simulink model "gm_mandelbrot_fpga"  (R2019b)
settings: Solver=FixedStepDiscrete  StartTime=0.0  StopTime=33.5e-3  FixedStep=0.5*Ts  RelTol=1e-3  EnableMultiTasking=on
undefined symbols (not defined in the file or in its folder): BUTTON_CLOCK_DIV, BUTTON_DEBOUNCE, BUTTON_POLLING, LUT_BLUE, LUT_GREEN, LUT_RED, MAX_ITERATIONS, PIXEL_TIME, TRASLATION_FACTOR, Ts, VGA_HORIZONTAL_BACK_PORCH, VGA_HORIZONTAL_FRONT_PORCH, VGA_HORIZONTAL_RESOLUTION, VGA_HORIZONTAL_SYNC, VGA_VERTICAL_BACK_PORCH, VGA_VERTICAL_FRONT_PORCH, VGA_VERTICAL_RESOLUTION, VGA_VERTICAL_SYNC, ZOOM_FACTOR
libraries: simulink x132, hdlsllib x20, visionsinks x1
(part 2 of 9)

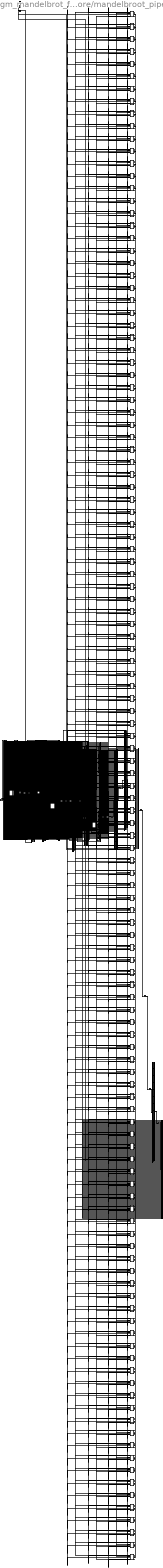
== system gm_mandelbrot_fpga/mandelbrot_top/mandelbrot_core/mandelbroot_pipeline ==
  c : Inport  OutDataTypeStr=fixdt(1, 18, 15)  PortDimensions=1  SampleTime=1.35e-08
      settings: SignalType=complex
  Constant : Constant  Value=0  OutDataTypeStr=boolean  SampleTime=-1
  Constant2 : Constant  Value=127  OutDataTypeStr=fixdt(0, 7, 0)  SampleTime=-1
  Delay{,1..3} (4 alike) : Delay  DelayLength=double(1)  InitialCondition=0  SampleTime=1.35e-08
  Demux1_mux_1 : Mux  Inputs=127
  Demux2_mux_1 : Mux  Inputs=127
  Demux3_mux_1 : Mux  Inputs=127
  Demux_mux_1 : Mux  Inputs=127
  Signal Specification : SignalSpecification  OutDataTypeStr=boolean  Dimensions=128
  Signal Specification1 : SignalSpecification  OutDataTypeStr=fixdt(1, 18, 15)  Dimensions=128
  Signal Specification2 : SignalSpecification  OutDataTypeStr=fixdt(1, 18, 15)  Dimensions=128
  Signal Specification3 : SignalSpecification  OutDataTypeStr=fixdt(0, 7, 0)  Dimensions=128
  Signal Specification4 : SignalSpecification  OutDataTypeStr=boolean  Dimensions=127
  Signal Specification5 : SignalSpecification  OutDataTypeStr=fixdt(1, 18, 15)  Dimensions=127
  Signal Specification6 : SignalSpecification  OutDataTypeStr=fixdt(1, 18, 15)  Dimensions=127
  Signal Specification7 : SignalSpecification  OutDataTypeStr=fixdt(0, 7, 0)  Dimensions=127
  Terminator : Terminator
  Terminator1 : Terminator
  Terminator2 : Terminator
  concatenate{,1..3} (4 alike) : Concatenate  NumInputs=128
  mandelbroot_array_instance1 : Subsystem
  mandelbroot_array_instance10 : Subsystem
  mandelbroot_array_instance100 : Subsystem
  mandelbroot_array_instance101 : Subsystem
  mandelbroot_array_instance102 : Subsystem
  mandelbroot_array_instance103 : Subsystem
  mandelbroot_array_instance104 : Subsystem
  mandelbroot_array_instance105 : Subsystem
  mandelbroot_array_instance106 : Subsystem
  mandelbroot_array_instance107 : Subsystem
  mandelbroot_array_instance108 : Subsystem
  mandelbroot_array_instance109 : Subsystem
  mandelbroot_array_instance11 : Subsystem
  mandelbroot_array_instance110 : Subsystem
  mandelbroot_array_instance111 : Subsystem
  mandelbroot_array_instance112 : Subsystem
  mandelbroot_array_instance113 : Subsystem
  mandelbroot_array_instance114 : Subsystem
  mandelbroot_array_instance115 : Subsystem
  mandelbroot_array_instance116 : Subsystem
  mandelbroot_array_instance117 : Subsystem
  mandelbroot_array_instance118 : Subsystem
  mandelbroot_array_instance119 : Subsystem
  mandelbroot_array_instance12 : Subsystem
  mandelbroot_array_instance120 : Subsystem
  mandelbroot_array_instance121 : Subsystem
  mandelbroot_array_instance122 : Subsystem
  mandelbroot_array_instance123 : Subsystem
  mandelbroot_array_instance124 : Subsystem
  mandelbroot_array_instance125 : Subsystem
  mandelbroot_array_instance126 : Subsystem
  mandelbroot_array_instance127 : Subsystem
  mandelbroot_array_instance128 : Subsystem
  mandelbroot_array_instance13 : Subsystem
  mandelbroot_array_instance14 : Subsystem
  mandelbroot_array_instance15 : Subsystem
  mandelbroot_array_instance16 : Subsystem
  mandelbroot_array_instance17 : Subsystem
  mandelbroot_array_instance18 : Subsystem
  mandelbroot_array_instance19 : Subsystem
  mandelbroot_array_instance2 : Subsystem
  mandelbroot_array_instance20 : Subsystem
  mandelbroot_array_instance21 : Subsystem
  mandelbroot_array_instance22 : Subsystem
  mandelbroot_array_instance23 : Subsystem
  mandelbroot_array_instance24 : Subsystem
  mandelbroot_array_instance25 : Subsystem
  mandelbroot_array_instance26 : Subsystem
  mandelbroot_array_instance27 : Subsystem
  mandelbroot_array_instance28 : Subsystem
  mandelbroot_array_instance29 : Subsystem
  mandelbroot_array_instance3 : Subsystem
  mandelbroot_array_instance30 : Subsystem
  mandelbroot_array_instance31 : Subsystem
  mandelbroot_array_instance32 : Subsystem
  mandelbroot_array_instance33 : Subsystem
  mandelbroot_array_instance34 : Subsystem
  mandelbroot_array_instance35 : Subsystem
  mandelbroot_array_instance36 : Subsystem
  mandelbroot_array_instance37 : Subsystem
  mandelbroot_array_instance38 : Subsystem
  mandelbroot_array_instance39 : Subsystem
  mandelbroot_array_instance4 : Subsystem
  mandelbroot_array_instance40 : Subsystem
  mandelbroot_array_instance41 : Subsystem
  mandelbroot_array_instance42 : Subsystem
  mandelbroot_array_instance43 : Subsystem
  mandelbroot_array_instance44 : Subsystem
  mandelbroot_array_instance45 : Subsystem
  mandelbroot_array_instance46 : Subsystem
  mandelbroot_array_instance47 : Subsystem
  mandelbroot_array_instance48 : Subsystem
  mandelbroot_array_instance49 : Subsystem
  mandelbroot_array_instance5 : Subsystem
  mandelbroot_array_instance50 : Subsystem
  mandelbroot_array_instance51 : Subsystem
  mandelbroot_array_instance52 : Subsystem
  mandelbroot_array_instance53 : Subsystem
  mandelbroot_array_instance54 : Subsystem
  mandelbroot_array_instance55 : Subsystem
  mandelbroot_array_instance56 : Subsystem
  mandelbroot_array_instance57 : Subsystem
  mandelbroot_array_instance58 : Subsystem
  mandelbroot_array_instance59 : Subsystem
  mandelbroot_array_instance6 : Subsystem
  mandelbroot_array_instance60 : Subsystem
  mandelbroot_array_instance61 : Subsystem
  mandelbroot_array_instance62 : Subsystem
  mandelbroot_array_instance63 : Subsystem
  mandelbroot_array_instance64 : Subsystem
  mandelbroot_array_instance65 : Subsystem
  mandelbroot_array_instance66 : Subsystem
  mandelbroot_array_instance67 : Subsystem
  mandelbroot_array_instance68 : Subsystem
  mandelbroot_array_instance69 : Subsystem
  mandelbroot_array_instance7 : Subsystem
  mandelbroot_array_instance70 : Subsystem
  mandelbroot_array_instance71 : Subsystem
  mandelbroot_array_instance72 : Subsystem
  mandelbroot_array_instance73 : Subsystem
  mandelbroot_array_instance74 : Subsystem
  mandelbroot_array_instance75 : Subsystem
  mandelbroot_array_instance76 : Subsystem
  mandelbroot_array_instance77 : Subsystem
  mandelbroot_array_instance78 : Subsystem
  mandelbroot_array_instance79 : Subsystem
  mandelbroot_array_instance8 : Subsystem
  mandelbroot_array_instance80 : Subsystem
  mandelbroot_array_instance81 : Subsystem
  mandelbroot_array_instance82 : Subsystem
  mandelbroot_array_instance83 : Subsystem
  mandelbroot_array_instance84 : Subsystem
  mandelbroot_array_instance85 : Subsystem
  mandelbroot_array_instance86 : Subsystem
  mandelbroot_array_instance87 : Subsystem
  mandelbroot_array_instance88 : Subsystem
  mandelbroot_array_instance89 : Subsystem
  mandelbroot_array_instance9 : Subsystem
  mandelbroot_array_instance90 : Subsystem
  mandelbroot_array_instance91 : Subsystem
  mandelbroot_array_instance92 : Subsystem
  mandelbroot_array_instance93 : Subsystem
  mandelbroot_array_instance94 : Subsystem
  mandelbroot_array_instance95 : Subsystem
  mandelbroot_array_instance96 : Subsystem
  mandelbroot_array_instance97 : Subsystem
  mandelbroot_array_instance98 : Subsystem
  mandelbroot_array_instance99 : Subsystem
  t{,1..3,12..15} (8 alike) : Demux  Outputs=128
  t{4,6,8,10} (4 alike) : Concatenate  NumInputs=128
  t{5,7,9,11} (4 alike) : Reshape
  t{16..19} (4 alike) : Demux  Outputs=127
  result : Outport  VectorParamsAs1DForOutWhenUnconnected=off
  wires:
  c/1 -> concatenate2/1, concatenate/1
  Constant/1 -> concatenate1/1
  Constant2/1 -> concatenate3/1
  Delay/1 -> Signal Specification/1
  Delay1/1 -> Signal Specification1/1
  Delay2/1 -> Signal Specification3/1
  Delay3/1 -> Signal Specification2/1
  Demux_mux_1/1 -> Signal Specification4/1
  Demux1_mux_1/1 -> Signal Specification5/1
  Demux2_mux_1/1 -> Signal Specification6/1
  Demux3_mux_1/1 -> Signal Specification7/1
  Signal Specification/1 -> t12/1
  Signal Specification1/1 -> t13/1
  Signal Specification2/1 -> t14/1
  Signal Specification3/1 -> t15/1
  Signal Specification4/1 -> t17/1
  Signal Specification5/1 -> t18/1
  Signal Specification6/1 -> t16/1
  Signal Specification7/1 -> t19/1
  concatenate/1 -> t2/1
  concatenate1/1 -> t/1
  concatenate2/1 -> t1/1
  concatenate3/1 -> t3/1
  t5/1 -> Delay/1
  t7/1 -> Delay1/1
  t9/1 -> Delay3/1
  t11/1 -> Delay2/1
  t/1 -> mandelbroot_array_instance1/1(stop_in)
  t/2 -> mandelbroot_array_instance2/1(stop_in)
  t/3 -> mandelbroot_array_instance3/1(stop_in)
  t/4 -> mandelbroot_array_instance4/1(stop_in)
  t/5 -> mandelbroot_array_instance5/1(stop_in)
  t/6 -> mandelbroot_array_instance6/1(stop_in)
  t/7 -> mandelbroot_array_instance7/1(stop_in)
  t/8 -> mandelbroot_array_instance8/1(stop_in)
  t/9 -> mandelbroot_array_instance9/1(stop_in)
  t/10 -> mandelbroot_array_instance10/1(stop_in)
  t/11 -> mandelbroot_array_instance11/1(stop_in)
  t/12 -> mandelbroot_array_instance12/1(stop_in)
  t/13 -> mandelbroot_array_instance13/1(stop_in)
  t/14 -> mandelbroot_array_instance14/1(stop_in)
  t/15 -> mandelbroot_array_instance15/1(stop_in)
  t/16 -> mandelbroot_array_instance16/1(stop_in)
  t/17 -> mandelbroot_array_instance17/1(stop_in)
  t/18 -> mandelbroot_array_instance18/1(stop_in)
  t/19 -> mandelbroot_array_instance19/1(stop_in)
  t/20 -> mandelbroot_array_instance20/1(stop_in)
  t/21 -> mandelbroot_array_instance21/1(stop_in)
  t/22 -> mandelbroot_array_instance22/1(stop_in)
  t/23 -> mandelbroot_array_instance23/1(stop_in)
  t/24 -> mandelbroot_array_instance24/1(stop_in)
  t/25 -> mandelbroot_array_instance25/1(stop_in)
  t/26 -> mandelbroot_array_instance26/1(stop_in)
  t/27 -> mandelbroot_array_instance27/1(stop_in)
  t/28 -> mandelbroot_array_instance28/1(stop_in)
  t/29 -> mandelbroot_array_instance29/1(stop_in)
  t/30 -> mandelbroot_array_instance30/1(stop_in)
  t/31 -> mandelbroot_array_instance31/1(stop_in)
  t/32 -> mandelbroot_array_instance32/1(stop_in)
  t/33 -> mandelbroot_array_instance33/1(stop_in)
  t/34 -> mandelbroot_array_instance34/1(stop_in)
  t/35 -> mandelbroot_array_instance35/1(stop_in)
  t/36 -> mandelbroot_array_instance36/1(stop_in)
  t/37 -> mandelbroot_array_instance37/1(stop_in)
  t/38 -> mandelbroot_array_instance38/1(stop_in)
  t/39 -> mandelbroot_array_instance39/1(stop_in)
  t/40 -> mandelbroot_array_instance40/1(stop_in)
  t/41 -> mandelbroot_array_instance41/1(stop_in)
  t/42 -> mandelbroot_array_instance42/1(stop_in)
  t/43 -> mandelbroot_array_instance43/1(stop_in)
  t/44 -> mandelbroot_array_instance44/1(stop_in)
  t/45 -> mandelbroot_array_instance45/1(stop_in)
  t/46 -> mandelbroot_array_instance46/1(stop_in)
  t/47 -> mandelbroot_array_instance47/1(stop_in)
  t/48 -> mandelbroot_array_instance48/1(stop_in)
  t/49 -> mandelbroot_array_instance49/1(stop_in)
  t/50 -> mandelbroot_array_instance50/1(stop_in)
  t/51 -> mandelbroot_array_instance51/1(stop_in)
  t/52 -> mandelbroot_array_instance52/1(stop_in)
  t/53 -> mandelbroot_array_instance53/1(stop_in)
  t/54 -> mandelbroot_array_instance54/1(stop_in)
  t/55 -> mandelbroot_array_instance55/1(stop_in)
  t/56 -> mandelbroot_array_instance56/1(stop_in)
  t/57 -> mandelbroot_array_instance57/1(stop_in)
  t/58 -> mandelbroot_array_instance58/1(stop_in)
  t/59 -> mandelbroot_array_instance59/1(stop_in)
  t/60 -> mandelbroot_array_instance60/1(stop_in)
  t/61 -> mandelbroot_array_instance61/1(stop_in)
  t/62 -> mandelbroot_array_instance62/1(stop_in)
  t/63 -> mandelbroot_array_instance63/1(stop_in)
  t/64 -> mandelbroot_array_instance64/1(stop_in)
  t/65 -> mandelbroot_array_instance65/1(stop_in)
  t/66 -> mandelbroot_array_instance66/1(stop_in)
  t/67 -> mandelbroot_array_instance67/1(stop_in)
  t/68 -> mandelbroot_array_instance68/1(stop_in)
  t/69 -> mandelbroot_array_instance69/1(stop_in)
  t/70 -> mandelbroot_array_instance70/1(stop_in)
  t/71 -> mandelbroot_array_instance71/1(stop_in)
  t/72 -> mandelbroot_array_instance72/1(stop_in)
  t/73 -> mandelbroot_array_instance73/1(stop_in)
  t/74 -> mandelbroot_array_instance74/1(stop_in)
  t/75 -> mandelbroot_array_instance75/1(stop_in)
  t/76 -> mandelbroot_array_instance76/1(stop_in)
  t/77 -> mandelbroot_array_instance77/1(stop_in)
  t/78 -> mandelbroot_array_instance78/1(stop_in)
  t/79 -> mandelbroot_array_instance79/1(stop_in)
  t/80 -> mandelbroot_array_instance80/1(stop_in)
  t/81 -> mandelbroot_array_instance81/1(stop_in)
  t/82 -> mandelbroot_array_instance82/1(stop_in)
  t/83 -> mandelbroot_array_instance83/1(stop_in)
  t/84 -> mandelbroot_array_instance84/1(stop_in)
  t/85 -> mandelbroot_array_instance85/1(stop_in)
  t/86 -> mandelbroot_array_instance86/1(stop_in)
  t/87 -> mandelbroot_array_instance87/1(stop_in)
  t/88 -> mandelbroot_array_instance88/1(stop_in)
  t/89 -> mandelbroot_array_instance89/1(stop_in)
  t/90 -> mandelbroot_array_instance90/1(stop_in)
  t/91 -> mandelbroot_array_instance91/1(stop_in)
  t/92 -> mandelbroot_array_instance92/1(stop_in)
  t/93 -> mandelbroot_array_instance93/1(stop_in)
  t/94 -> mandelbroot_array_instance94/1(stop_in)
  t/95 -> mandelbroot_array_instance95/1(stop_in)
  t/96 -> mandelbroot_array_instance96/1(stop_in)
  t/97 -> mandelbroot_array_instance97/1(stop_in)
  t/98 -> mandelbroot_array_instance98/1(stop_in)
  t/99 -> mandelbroot_array_instance99/1(stop_in)
  t/100 -> mandelbroot_array_instance100/1(stop_in)
  t/101 -> mandelbroot_array_instance101/1(stop_in)
  t/102 -> mandelbroot_array_instance102/1(stop_in)
  t/103 -> mandelbroot_array_instance103/1(stop_in)
  t/104 -> mandelbroot_array_instance104/1(stop_in)
  t/105 -> mandelbroot_array_instance105/1(stop_in)
  t/106 -> mandelbroot_array_instance106/1(stop_in)
  t/107 -> mandelbroot_array_instance107/1(stop_in)
  t/108 -> mandelbroot_array_instance108/1(stop_in)
  t/109 -> mandelbroot_array_instance109/1(stop_in)
  t/110 -> mandelbroot_array_instance110/1(stop_in)
  t/111 -> mandelbroot_array_instance111/1(stop_in)
  t/112 -> mandelbroot_array_instance112/1(stop_in)
  t/113 -> mandelbroot_array_instance113/1(stop_in)
  t/114 -> mandelbroot_array_instance114/1(stop_in)
  t/115 -> mandelbroot_array_instance115/1(stop_in)
  t/116 -> mandelbroot_array_instance116/1(stop_in)
  t/117 -> mandelbroot_array_instance117/1(stop_in)
  t/118 -> mandelbroot_array_instance118/1(stop_in)
  t/119 -> mandelbroot_array_instance119/1(stop_in)
  t/120 -> mandelbroot_array_instance120/1(stop_in)
  t/121 -> mandelbroot_array_instance121/1(stop_in)
  t/122 -> mandelbroot_array_instance122/1(stop_in)
  t/123 -> mandelbroot_array_instance123/1(stop_in)
  t/124 -> mandelbroot_array_instance124/1(stop_in)
  t/125 -> mandelbroot_array_instance125/1(stop_in)
  t/126 -> mandelbroot_array_instance126/1(stop_in)
  t/127 -> mandelbroot_array_instance127/1(stop_in)
  t/128 -> mandelbroot_array_instance128/1(stop_in)
  t1/1 -> mandelbroot_array_instance1/2(z_in)
  t1/2 -> mandelbroot_array_instance2/2(z_in)
  t1/3 -> mandelbroot_array_instance3/2(z_in)
  t1/4 -> mandelbroot_array_instance4/2(z_in)
  t1/5 -> mandelbroot_array_instance5/2(z_in)
  t1/6 -> mandelbroot_array_instance6/2(z_in)
  t1/7 -> mandelbroot_array_instance7/2(z_in)
  t1/8 -> mandelbroot_array_instance8/2(z_in)
  t1/9 -> mandelbroot_array_instance9/2(z_in)
  t1/10 -> mandelbroot_array_instance10/2(z_in)
  t1/11 -> mandelbroot_array_instance11/2(z_in)
  t1/12 -> mandelbroot_array_instance12/2(z_in)
  t1/13 -> mandelbroot_array_instance13/2(z_in)
  t1/14 -> mandelbroot_array_instance14/2(z_in)
  t1/15 -> mandelbroot_array_instance15/2(z_in)
  t1/16 -> mandelbroot_array_instance16/2(z_in)
  t1/17 -> mandelbroot_array_instance17/2(z_in)
  t1/18 -> mandelbroot_array_instance18/2(z_in)
  t1/19 -> mandelbroot_array_instance19/2(z_in)
  t1/20 -> mandelbroot_array_instance20/2(z_in)
  t1/21 -> mandelbroot_array_instance21/2(z_in)
  t1/22 -> mandelbroot_array_instance22/2(z_in)
  t1/23 -> mandelbroot_array_instance23/2(z_in)
  t1/24 -> mandelbroot_array_instance24/2(z_in)
  t1/25 -> mandelbroot_array_instance25/2(z_in)
  t1/26 -> mandelbroot_array_instance26/2(z_in)
  t1/27 -> mandelbroot_array_instance27/2(z_in)
  t1/28 -> mandelbroot_array_instance28/2(z_in)
  t1/29 -> mandelbroot_array_instance29/2(z_in)
  t1/30 -> mandelbroot_array_instance30/2(z_in)
  t1/31 -> mandelbroot_array_instance31/2(z_in)
  t1/32 -> mandelbroot_array_instance32/2(z_in)
  t1/33 -> mandelbroot_array_instance33/2(z_in)
  t1/34 -> mandelbroot_array_instance34/2(z_in)
  t1/35 -> mandelbroot_array_instance35/2(z_in)
  t1/36 -> mandelbroot_array_instance36/2(z_in)
  t1/37 -> mandelbroot_array_instance37/2(z_in)
  t1/38 -> mandelbroot_array_instance38/2(z_in)
  t1/39 -> mandelbroot_array_instance39/2(z_in)
  t1/40 -> mandelbroot_array_instance40/2(z_in)
  t1/41 -> mandelbroot_array_instance41/2(z_in)
  t1/42 -> mandelbroot_array_instance42/2(z_in)
  t1/43 -> mandelbroot_array_instance43/2(z_in)
  t1/44 -> mandelbroot_array_instance44/2(z_in)
  t1/45 -> mandelbroot_array_instance45/2(z_in)
  t1/46 -> mandelbroot_array_instance46/2(z_in)
  t1/47 -> mandelbroot_array_instance47/2(z_in)
  t1/48 -> mandelbroot_array_instance48/2(z_in)
  t1/49 -> mandelbroot_array_instance49/2(z_in)
  t1/50 -> mandelbroot_array_instance50/2(z_in)
  t1/51 -> mandelbroot_array_instance51/2(z_in)
  t1/52 -> mandelbroot_array_instance52/2(z_in)
  t1/53 -> mandelbroot_array_instance53/2(z_in)
  t1/54 -> mandelbroot_array_instance54/2(z_in)
  t1/55 -> mandelbroot_array_instance55/2(z_in)
  t1/56 -> mandelbroot_array_instance56/2(z_in)
  t1/57 -> mandelbroot_array_instance57/2(z_in)
  t1/58 -> mandelbroot_array_instance58/2(z_in)
  t1/59 -> mandelbroot_array_instance59/2(z_in)
  t1/60 -> mandelbroot_array_instance60/2(z_in)
  t1/61 -> mandelbroot_array_instance61/2(z_in)
  t1/62 -> mandelbroot_array_instance62/2(z_in)
  t1/63 -> mandelbroot_array_instance63/2(z_in)
  t1/64 -> mandelbroot_array_instance64/2(z_in)
  t1/65 -> mandelbroot_array_instance65/2(z_in)
  t1/66 -> mandelbroot_array_instance66/2(z_in)
  t1/67 -> mandelbroot_array_instance67/2(z_in)
  t1/68 -> mandelbroot_array_instance68/2(z_in)
  t1/69 -> mandelbroot_array_instance69/2(z_in)
  t1/70 -> mandelbroot_array_instance70/2(z_in)
  t1/71 -> mandelbroot_array_instance71/2(z_in)
  t1/72 -> mandelbroot_array_instance72/2(z_in)
  t1/73 -> mandelbroot_array_instance73/2(z_in)
  t1/74 -> mandelbroot_array_instance74/2(z_in)
  t1/75 -> mandelbroot_array_instance75/2(z_in)
  t1/76 -> mandelbroot_array_instance76/2(z_in)
  t1/77 -> mandelbroot_array_instance77/2(z_in)
  t1/78 -> mandelbroot_array_instance78/2(z_in)
  t1/79 -> mandelbroot_array_instance79/2(z_in)
  t1/80 -> mandelbroot_array_instance80/2(z_in)
  t1/81 -> mandelbroot_array_instance81/2(z_in)
  t1/82 -> mandelbroot_array_instance82/2(z_in)
  t1/83 -> mandelbroot_array_instance83/2(z_in)
  t1/84 -> mandelbroot_array_instance84/2(z_in)
  t1/85 -> mandelbroot_array_instance85/2(z_in)
  t1/86 -> mandelbroot_array_instance86/2(z_in)
  t1/87 -> mandelbroot_array_instance87/2(z_in)
  t1/88 -> mandelbroot_array_instance88/2(z_in)
  t1/89 -> mandelbroot_array_instance89/2(z_in)
  t1/90 -> mandelbroot_array_instance90/2(z_in)
  t1/91 -> mandelbroot_array_instance91/2(z_in)
  t1/92 -> mandelbroot_array_instance92/2(z_in)
  t1/93 -> mandelbroot_array_instance93/2(z_in)
  t1/94 -> mandelbroot_array_instance94/2(z_in)
  t1/95 -> mandelbroot_array_instance95/2(z_in)
  t1/96 -> mandelbroot_array_instance96/2(z_in)
  t1/97 -> mandelbroot_array_instance97/2(z_in)
  t1/98 -> mandelbroot_array_instance98/2(z_in)
  t1/99 -> mandelbroot_array_instance99/2(z_in)
  t1/100 -> mandelbroot_array_instance100/2(z_in)
  t1/101 -> mandelbroot_array_instance101/2(z_in)
  t1/102 -> mandelbroot_array_instance102/2(z_in)
  t1/103 -> mandelbroot_array_instance103/2(z_in)
  t1/104 -> mandelbroot_array_instance104/2(z_in)
  t1/105 -> mandelbroot_array_instance105/2(z_in)
  t1/106 -> mandelbroot_array_instance106/2(z_in)
  t1/107 -> mandelbroot_array_instance107/2(z_in)
  t1/108 -> mandelbroot_array_instance108/2(z_in)
  t1/109 -> mandelbroot_array_instance109/2(z_in)
  t1/110 -> mandelbroot_array_instance110/2(z_in)
  t1/111 -> mandelbroot_array_instance111/2(z_in)
  t1/112 -> mandelbroot_array_instance112/2(z_in)
  t1/113 -> mandelbroot_array_instance113/2(z_in)
  t1/114 -> mandelbroot_array_instance114/2(z_in)
  t1/115 -> mandelbroot_array_instance115/2(z_in)
  t1/116 -> mandelbroot_array_instance116/2(z_in)
  t1/117 -> mandelbroot_array_instance117/2(z_in)
  t1/118 -> mandelbroot_array_instance118/2(z_in)
  t1/119 -> mandelbroot_array_instance119/2(z_in)
  t1/120 -> mandelbroot_array_instance120/2(z_in)
  t1/121 -> mandelbroot_array_instance121/2(z_in)
  t1/122 -> mandelbroot_array_instance122/2(z_in)
  t1/123 -> mandelbroot_array_instance123/2(z_in)
  t1/124 -> mandelbroot_array_instance124/2(z_in)
  t1/125 -> mandelbroot_array_instance125/2(z_in)
  t1/126 -> mandelbroot_array_instance126/2(z_in)
  t1/127 -> mandelbroot_array_instance127/2(z_in)
  t1/128 -> mandelbroot_array_instance128/2(z_in)
  t2/1 -> mandelbroot_array_instance1/3(c_in)
  t2/2 -> mandelbroot_array_instance2/3(c_in)
  t2/3 -> mandelbroot_array_instance3/3(c_in)
  t2/4 -> mandelbroot_array_instance4/3(c_in)
  t2/5 -> mandelbroot_array_instance5/3(c_in)
  t2/6 -> mandelbroot_array_instance6/3(c_in)
  t2/7 -> mandelbroot_array_instance7/3(c_in)
  t2/8 -> mandelbroot_array_instance8/3(c_in)
  t2/9 -> mandelbroot_array_instance9/3(c_in)
  t2/10 -> mandelbroot_array_instance10/3(c_in)
  t2/11 -> mandelbroot_array_instance11/3(c_in)
  t2/12 -> mandelbroot_array_instance12/3(c_in)
  t2/13 -> mandelbroot_array_instance13/3(c_in)
  t2/14 -> mandelbroot_array_instance14/3(c_in)
  t2/15 -> mandelbroot_array_instance15/3(c_in)
  t2/16 -> mandelbroot_array_instance16/3(c_in)
  t2/17 -> mandelbroot_array_instance17/3(c_in)
  t2/18 -> mandelbroot_array_instance18/3(c_in)
  t2/19 -> mandelbroot_array_instance19/3(c_in)
  t2/20 -> mandelbroot_array_instance20/3(c_in)
  t2/21 -> mandelbroot_array_instance21/3(c_in)
  t2/22 -> mandelbroot_array_instance22/3(c_in)
  t2/23 -> mandelbroot_array_instance23/3(c_in)
  t2/24 -> mandelbroot_array_instance24/3(c_in)
  t2/25 -> mandelbroot_array_instance25/3(c_in)
  t2/26 -> mandelbroot_array_instance26/3(c_in)
  t2/27 -> mandelbroot_array_instance27/3(c_in)
  t2/28 -> mandelbroot_array_instance28/3(c_in)
  t2/29 -> mandelbroot_array_instance29/3(c_in)
  t2/30 -> mandelbroot_array_instance30/3(c_in)
  t2/31 -> mandelbroot_array_instance31/3(c_in)
  t2/32 -> mandelbroot_array_instance32/3(c_in)
  t2/33 -> mandelbroot_array_instance33/3(c_in)
  t2/34 -> mandelbroot_array_instance34/3(c_in)
  t2/35 -> mandelbroot_array_instance35/3(c_in)
  t2/36 -> mandelbroot_array_instance36/3(c_in)
  t2/37 -> mandelbroot_array_instance37/3(c_in)
  t2/38 -> mandelbroot_array_instance38/3(c_in)
  t2/39 -> mandelbroot_array_instance39/3(c_in)
  t2/40 -> mandelbroot_array_instance40/3(c_in)
  t2/41 -> mandelbroot_array_instance41/3(c_in)
  t2/42 -> mandelbroot_array_instance42/3(c_in)
  t2/43 -> mandelbroot_array_instance43/3(c_in)
  t2/44 -> mandelbroot_array_instance44/3(c_in)
  t2/45 -> mandelbroot_array_instance45/3(c_in)
  t2/46 -> mandelbroot_array_instance46/3(c_in)
  t2/47 -> mandelbroot_array_instance47/3(c_in)
  t2/48 -> mandelbroot_array_instance48/3(c_in)
  t2/49 -> mandelbroot_array_instance49/3(c_in)
  t2/50 -> mandelbroot_array_instance50/3(c_in)
  t2/51 -> mandelbroot_array_instance51/3(c_in)
  t2/52 -> mandelbroot_array_instance52/3(c_in)
  t2/53 -> mandelbroot_array_instance53/3(c_in)
  t2/54 -> mandelbroot_array_instance54/3(c_in)
  t2/55 -> mandelbroot_array_instance55/3(c_in)
  t2/56 -> mandelbroot_array_instance56/3(c_in)
  t2/57 -> mandelbroot_array_instance57/3(c_in)
  t2/58 -> mandelbroot_array_instance58/3(c_in)
  t2/59 -> mandelbroot_array_instance59/3(c_in)
  t2/60 -> mandelbroot_array_instance60/3(c_in)
  t2/61 -> mandelbroot_array_instance61/3(c_in)
  t2/62 -> mandelbroot_array_instance62/3(c_in)
  t2/63 -> mandelbroot_array_instance63/3(c_in)
  t2/64 -> mandelbroot_array_instance64/3(c_in)
  t2/65 -> mandelbroot_array_instance65/3(c_in)
  t2/66 -> mandelbroot_array_instance66/3(c_in)
  t2/67 -> mandelbroot_array_instance67/3(c_in)
  t2/68 -> mandelbroot_array_instance68/3(c_in)
  t2/69 -> mandelbroot_array_instance69/3(c_in)
  t2/70 -> mandelbroot_array_instance70/3(c_in)
  t2/71 -> mandelbroot_array_instance71/3(c_in)
  t2/72 -> mandelbroot_array_instance72/3(c_in)
  t2/73 -> mandelbroot_array_instance73/3(c_in)
  t2/74 -> mandelbroot_array_instance74/3(c_in)
  t2/75 -> mandelbroot_array_instance75/3(c_in)
  t2/76 -> mandelbroot_array_instance76/3(c_in)
  t2/77 -> mandelbroot_array_instance77/3(c_in)
  t2/78 -> mandelbroot_array_instance78/3(c_in)
  t2/79 -> mandelbroot_array_instance79/3(c_in)
  t2/80 -> mandelbroot_array_instance80/3(c_in)
  t2/81 -> mandelbroot_array_instance81/3(c_in)
  t2/82 -> mandelbroot_array_instance82/3(c_in)
  t2/83 -> mandelbroot_array_instance83/3(c_in)
  t2/84 -> mandelbroot_array_instance84/3(c_in)
  t2/85 -> mandelbroot_array_instance85/3(c_in)
  t2/86 -> mandelbroot_array_instance86/3(c_in)
  t2/87 -> mandelbroot_array_instance87/3(c_in)
  t2/88 -> mandelbroot_array_instance88/3(c_in)
  t2/89 -> mandelbroot_array_instance89/3(c_in)
  t2/90 -> mandelbroot_array_instance90/3(c_in)
  t2/91 -> mandelbroot_array_instance91/3(c_in)
  t2/92 -> mandelbroot_array_instance92/3(c_in)
  t2/93 -> mandelbroot_array_instance93/3(c_in)
  t2/94 -> mandelbroot_array_instance94/3(c_in)
  t2/95 -> mandelbroot_array_instance95/3(c_in)
  t2/96 -> mandelbroot_array_instance96/3(c_in)
  t2/97 -> mandelbroot_array_instance97/3(c_in)
  t2/98 -> mandelbroot_array_instance98/3(c_in)
  t2/99 -> mandelbroot_array_instance99/3(c_in)
  t2/100 -> mandelbroot_array_instance100/3(c_in)
  t2/101 -> mandelbroot_array_instance101/3(c_in)
  t2/102 -> mandelbroot_array_instance102/3(c_in)
  t2/103 -> mandelbroot_array_instance103/3(c_in)
  t2/104 -> mandelbroot_array_instance104/3(c_in)
  t2/105 -> mandelbroot_array_instance105/3(c_in)
  t2/106 -> mandelbroot_array_instance106/3(c_in)
  t2/107 -> mandelbroot_array_instance107/3(c_in)
  t2/108 -> mandelbroot_array_instance108/3(c_in)
  t2/109 -> mandelbroot_array_instance109/3(c_in)
  t2/110 -> mandelbroot_array_instance110/3(c_in)
  t2/111 -> mandelbroot_array_instance111/3(c_in)
  t2/112 -> mandelbroot_array_instance112/3(c_in)
  t2/113 -> mandelbroot_array_instance113/3(c_in)
  t2/114 -> mandelbroot_array_instance114/3(c_in)
  t2/115 -> mandelbroot_array_instance115/3(c_in)
  t2/116 -> mandelbroot_array_instance116/3(c_in)
  t2/117 -> mandelbroot_array_instance117/3(c_in)
  t2/118 -> mandelbroot_array_instance118/3(c_in)
  t2/119 -> mandelbroot_array_instance119/3(c_in)
  t2/120 -> mandelbroot_array_instance120/3(c_in)
  t2/121 -> mandelbroot_array_instance121/3(c_in)
  t2/122 -> mandelbroot_array_instance122/3(c_in)
  t2/123 -> mandelbroot_array_instance123/3(c_in)
  t2/124 -> mandelbroot_array_instance124/3(c_in)
  t2/125 -> mandelbroot_array_instance125/3(c_in)
  t2/126 -> mandelbroot_array_instance126/3(c_in)
  t2/127 -> mandelbroot_array_instance127/3(c_in)
  t2/128 -> mandelbroot_array_instance128/3(c_in)
  t3/1 -> mandelbroot_array_instance1/4(i_in)
  t3/2 -> mandelbroot_array_instance2/4(i_in)
  t3/3 -> mandelbroot_array_instance3/4(i_in)
  t3/4 -> mandelbroot_array_instance4/4(i_in)
  t3/5 -> mandelbroot_array_instance5/4(i_in)
  t3/6 -> mandelbroot_array_instance6/4(i_in)
  t3/7 -> mandelbroot_array_instance7/4(i_in)
  t3/8 -> mandelbroot_array_instance8/4(i_in)
  t3/9 -> mandelbroot_array_instance9/4(i_in)
  t3/10 -> mandelbroot_array_instance10/4(i_in)
  t3/11 -> mandelbroot_array_instance11/4(i_in)
  t3/12 -> mandelbroot_array_instance12/4(i_in)
  t3/13 -> mandelbroot_array_instance13/4(i_in)
  t3/14 -> mandelbroot_array_instance14/4(i_in)
  t3/15 -> mandelbroot_array_instance15/4(i_in)
  t3/16 -> mandelbroot_array_instance16/4(i_in)
  t3/17 -> mandelbroot_array_instance17/4(i_in)
  t3/18 -> mandelbroot_array_instance18/4(i_in)
  t3/19 -> mandelbroot_array_instance19/4(i_in)
  t3/20 -> mandelbroot_array_instance20/4(i_in)
  t3/21 -> mandelbroot_array_instance21/4(i_in)
  t3/22 -> mandelbroot_array_instance22/4(i_in)
  t3/23 -> mandelbroot_array_instance23/4(i_in)
  t3/24 -> mandelbroot_array_instance24/4(i_in)
  t3/25 -> mandelbroot_array_instance25/4(i_in)
  t3/26 -> mandelbroot_array_instance26/4(i_in)
  t3/27 -> mandelbroot_array_instance27/4(i_in)
  t3/28 -> mandelbroot_array_instance28/4(i_in)
  t3/29 -> mandelbroot_array_instance29/4(i_in)
  t3/30 -> mandelbroot_array_instance30/4(i_in)
  t3/31 -> mandelbroot_array_instance31/4(i_in)
  t3/32 -> mandelbroot_array_instance32/4(i_in)
  t3/33 -> mandelbroot_array_instance33/4(i_in)
  t3/34 -> mandelbroot_array_instance34/4(i_in)
  t3/35 -> mandelbroot_array_instance35/4(i_in)
  t3/36 -> mandelbroot_array_instance36/4(i_in)
  t3/37 -> mandelbroot_array_instance37/4(i_in)
  t3/38 -> mandelbroot_array_instance38/4(i_in)
  t3/39 -> mandelbroot_array_instance39/4(i_in)
  t3/40 -> mandelbroot_array_instance40/4(i_in)
  t3/41 -> mandelbroot_array_instance41/4(i_in)
  t3/42 -> mandelbroot_array_instance42/4(i_in)
  t3/43 -> mandelbroot_array_instance43/4(i_in)
  t3/44 -> mandelbroot_array_instance44/4(i_in)
  t3/45 -> mandelbroot_array_instance45/4(i_in)
  t3/46 -> mandelbroot_array_instance46/4(i_in)
  t3/47 -> mandelbroot_array_instance47/4(i_in)
  t3/48 -> mandelbroot_array_instance48/4(i_in)
  t3/49 -> mandelbroot_array_instance49/4(i_in)
  t3/50 -> mandelbroot_array_instance50/4(i_in)
  t3/51 -> mandelbroot_array_instance51/4(i_in)
  t3/52 -> mandelbroot_array_instance52/4(i_in)
  t3/53 -> mandelbroot_array_instance53/4(i_in)
  t3/54 -> mandelbroot_array_instance54/4(i_in)
  t3/55 -> mandelbroot_array_instance55/4(i_in)
  t3/56 -> mandelbroot_array_instance56/4(i_in)
  t3/57 -> mandelbroot_array_instance57/4(i_in)
  t3/58 -> mandelbroot_array_instance58/4(i_in)
  t3/59 -> mandelbroot_array_instance59/4(i_in)
  t3/60 -> mandelbroot_array_instance60/4(i_in)
  t3/61 -> mandelbroot_array_instance61/4(i_in)
  t3/62 -> mandelbroot_array_instance62/4(i_in)
  t3/63 -> mandelbroot_array_instance63/4(i_in)
  t3/64 -> mandelbroot_array_instance64/4(i_in)
  t3/65 -> mandelbroot_array_instance65/4(i_in)
  t3/66 -> mandelbroot_array_instance66/4(i_in)
  t3/67 -> mandelbroot_array_instance67/4(i_in)
  t3/68 -> mandelbroot_array_instance68/4(i_in)
  t3/69 -> mandelbroot_array_instance69/4(i_in)
  t3/70 -> mandelbroot_array_instance70/4(i_in)
  t3/71 -> mandelbroot_array_instance71/4(i_in)
  t3/72 -> mandelbroot_array_instance72/4(i_in)
  t3/73 -> mandelbroot_array_instance73/4(i_in)
  t3/74 -> mandelbroot_array_instance74/4(i_in)
  t3/75 -> mandelbroot_array_instance75/4(i_in)
  t3/76 -> mandelbroot_array_instance76/4(i_in)
  t3/77 -> mandelbroot_array_instance77/4(i_in)
  t3/78 -> mandelbroot_array_instance78/4(i_in)
  t3/79 -> mandelbroot_array_instance79/4(i_in)
  t3/80 -> mandelbroot_array_instance80/4(i_in)
  t3/81 -> mandelbroot_array_instance81/4(i_in)
  t3/82 -> mandelbroot_array_instance82/4(i_in)
  t3/83 -> mandelbroot_array_instance83/4(i_in)
  t3/84 -> mandelbroot_array_instance84/4(i_in)
  t3/85 -> mandelbroot_array_instance85/4(i_in)
  t3/86 -> mandelbroot_array_instance86/4(i_in)
  t3/87 -> mandelbroot_array_instance87/4(i_in)
  t3/88 -> mandelbroot_array_instance88/4(i_in)
  t3/89 -> mandelbroot_array_instance89/4(i_in)
  t3/90 -> mandelbroot_array_instance90/4(i_in)
  t3/91 -> mandelbroot_array_instance91/4(i_in)
  t3/92 -> mandelbroot_array_instance92/4(i_in)
  t3/93 -> mandelbroot_array_instance93/4(i_in)
  t3/94 -> mandelbroot_array_instance94/4(i_in)
  t3/95 -> mandelbroot_array_instance95/4(i_in)
  t3/96 -> mandelbroot_array_instance96/4(i_in)
  t3/97 -> mandelbroot_array_instance97/4(i_in)
  t3/98 -> mandelbroot_array_instance98/4(i_in)
  t3/99 -> mandelbroot_array_instance99/4(i_in)
  t3/100 -> mandelbroot_array_instance100/4(i_in)
  t3/101 -> mandelbroot_array_instance101/4(i_in)
  t3/102 -> mandelbroot_array_instance102/4(i_in)
  t3/103 -> mandelbroot_array_instance103/4(i_in)
  t3/104 -> mandelbroot_array_instance104/4(i_in)
  t3/105 -> mandelbroot_array_instance105/4(i_in)
  t3/106 -> mandelbroot_array_instance106/4(i_in)
  t3/107 -> mandelbroot_array_instance107/4(i_in)
  t3/108 -> mandelbroot_array_instance108/4(i_in)
  t3/109 -> mandelbroot_array_instance109/4(i_in)
  t3/110 -> mandelbroot_array_instance110/4(i_in)
  t3/111 -> mandelbroot_array_instance111/4(i_in)
  t3/112 -> mandelbroot_array_instance112/4(i_in)
  t3/113 -> mandelbroot_array_instance113/4(i_in)
  t3/114 -> mandelbroot_array_instance114/4(i_in)
  t3/115 -> mandelbroot_array_instance115/4(i_in)
  t3/116 -> mandelbroot_array_instance116/4(i_in)
  t3/117 -> mandelbroot_array_instance117/4(i_in)
  t3/118 -> mandelbroot_array_instance118/4(i_in)
  t3/119 -> mandelbroot_array_instance119/4(i_in)
  t3/120 -> mandelbroot_array_instance120/4(i_in)
  t3/121 -> mandelbroot_array_instance121/4(i_in)
  t3/122 -> mandelbroot_array_instance122/4(i_in)
  t3/123 -> mandelbroot_array_instance123/4(i_in)
  t3/124 -> mandelbroot_array_instance124/4(i_in)
  t3/125 -> mandelbroot_array_instance125/4(i_in)
  t3/126 -> mandelbroot_array_instance126/4(i_in)
  t3/127 -> mandelbroot_array_instance127/4(i_in)
  t3/128 -> mandelbroot_array_instance128/4(i_in)
  t4/1 -> t5/1
  mandelbroot_array_instance1/1(stop_out) -> t4/1
  mandelbroot_array_instance2/1(stop_out) -> t4/2
  mandelbroot_array_instance3/1(stop_out) -> t4/3
  mandelbroot_array_instance4/1(stop_out) -> t4/4
  mandelbroot_array_instance5/1(stop_out) -> t4/5
  mandelbroot_array_instance6/1(stop_out) -> t4/6
  mandelbroot_array_instance7/1(stop_out) -> t4/7
  mandelbroot_array_instance8/1(stop_out) -> t4/8
  mandelbroot_array_instance9/1(stop_out) -> t4/9
  mandelbroot_array_instance10/1(stop_out) -> t4/10
  mandelbroot_array_instance11/1(stop_out) -> t4/11
  mandelbroot_array_instance12/1(stop_out) -> t4/12
  mandelbroot_array_instance13/1(stop_out) -> t4/13
  mandelbroot_array_instance14/1(stop_out) -> t4/14
  mandelbroot_array_instance15/1(stop_out) -> t4/15
  mandelbroot_array_instance16/1(stop_out) -> t4/16
  mandelbroot_array_instance17/1(stop_out) -> t4/17
  mandelbroot_array_instance18/1(stop_out) -> t4/18
  mandelbroot_array_instance19/1(stop_out) -> t4/19
  mandelbroot_array_instance20/1(stop_out) -> t4/20
  mandelbroot_array_instance21/1(stop_out) -> t4/21
  mandelbroot_array_instance22/1(stop_out) -> t4/22
  mandelbroot_array_instance23/1(stop_out) -> t4/23
  mandelbroot_array_instance24/1(stop_out) -> t4/24
  mandelbroot_array_instance25/1(stop_out) -> t4/25
  mandelbroot_array_instance26/1(stop_out) -> t4/26
  mandelbroot_array_instance27/1(stop_out) -> t4/27
  mandelbroot_array_instance28/1(stop_out) -> t4/28
  mandelbroot_array_instance29/1(stop_out) -> t4/29
  mandelbroot_array_instance30/1(stop_out) -> t4/30
  mandelbroot_array_instance31/1(stop_out) -> t4/31
  mandelbroot_array_instance32/1(stop_out) -> t4/32
  mandelbroot_array_instance33/1(stop_out) -> t4/33
  mandelbroot_array_instance34/1(stop_out) -> t4/34
  mandelbroot_array_instance35/1(stop_out) -> t4/35
  mandelbroot_array_instance36/1(stop_out) -> t4/36
  mandelbroot_array_instance37/1(stop_out) -> t4/37
  mandelbroot_array_instance38/1(stop_out) -> t4/38
  mandelbroot_array_instance39/1(stop_out) -> t4/39
  mandelbroot_array_instance40/1(stop_out) -> t4/40
  mandelbroot_array_instance41/1(stop_out) -> t4/41
  mandelbroot_array_instance42/1(stop_out) -> t4/42
  mandelbroot_array_instance43/1(stop_out) -> t4/43
  mandelbroot_array_instance44/1(stop_out) -> t4/44
  mandelbroot_array_instance45/1(stop_out) -> t4/45
  mandelbroot_array_instance46/1(stop_out) -> t4/46
  mandelbroot_array_instance47/1(stop_out) -> t4/47
  mandelbroot_array_instance48/1(stop_out) -> t4/48
  mandelbroot_array_instance49/1(stop_out) -> t4/49
  mandelbroot_array_instance50/1(stop_out) -> t4/50
  mandelbroot_array_instance51/1(stop_out) -> t4/51
  mandelbroot_array_instance52/1(stop_out) -> t4/52
  mandelbroot_array_instance53/1(stop_out) -> t4/53
  mandelbroot_array_instance54/1(stop_out) -> t4/54
  mandelbroot_array_instance55/1(stop_out) -> t4/55
  mandelbroot_array_instance56/1(stop_out) -> t4/56
  mandelbroot_array_instance57/1(stop_out) -> t4/57
  mandelbroot_array_instance58/1(stop_out) -> t4/58
  mandelbroot_array_instance59/1(stop_out) -> t4/59
  mandelbroot_array_instance60/1(stop_out) -> t4/60
  mandelbroot_array_instance61/1(stop_out) -> t4/61
  mandelbroot_array_instance62/1(stop_out) -> t4/62
  mandelbroot_array_instance63/1(stop_out) -> t4/63
  mandelbroot_array_instance64/1(stop_out) -> t4/64
  mandelbroot_array_instance65/1(stop_out) -> t4/65
  mandelbroot_array_instance66/1(stop_out) -> t4/66
  mandelbroot_array_instance67/1(stop_out) -> t4/67
  mandelbroot_array_instance68/1(stop_out) -> t4/68
  mandelbroot_array_instance69/1(stop_out) -> t4/69
  mandelbroot_array_instance70/1(stop_out) -> t4/70
  mandelbroot_array_instance71/1(stop_out) -> t4/71
  mandelbroot_array_instance72/1(stop_out) -> t4/72
  mandelbroot_array_instance73/1(stop_out) -> t4/73
  mandelbroot_array_instance74/1(stop_out) -> t4/74
  mandelbroot_array_instance75/1(stop_out) -> t4/75
  mandelbroot_array_instance76/1(stop_out) -> t4/76
  mandelbroot_array_instance77/1(stop_out) -> t4/77
  mandelbroot_array_instance78/1(stop_out) -> t4/78
  mandelbroot_array_instance79/1(stop_out) -> t4/79
  mandelbroot_array_instance80/1(stop_out) -> t4/80
  mandelbroot_array_instance81/1(stop_out) -> t4/81
  mandelbroot_array_instance82/1(stop_out) -> t4/82
  mandelbroot_array_instance83/1(stop_out) -> t4/83
  mandelbroot_array_instance84/1(stop_out) -> t4/84
  mandelbroot_array_instance85/1(stop_out) -> t4/85
  mandelbroot_array_instance86/1(stop_out) -> t4/86
  mandelbroot_array_instance87/1(stop_out) -> t4/87
  mandelbroot_array_instance88/1(stop_out) -> t4/88
  mandelbroot_array_instance89/1(stop_out) -> t4/89
  mandelbroot_array_instance90/1(stop_out) -> t4/90
  mandelbroot_array_instance91/1(stop_out) -> t4/91
  mandelbroot_array_instance92/1(stop_out) -> t4/92
  mandelbroot_array_instance93/1(stop_out) -> t4/93
  mandelbroot_array_instance94/1(stop_out) -> t4/94
  mandelbroot_array_instance95/1(stop_out) -> t4/95
  mandelbroot_array_instance96/1(stop_out) -> t4/96
  mandelbroot_array_instance97/1(stop_out) -> t4/97
  mandelbroot_array_instance98/1(stop_out) -> t4/98
  mandelbroot_array_instance99/1(stop_out) -> t4/99
  mandelbroot_array_instance100/1(stop_out) -> t4/100
  mandelbroot_array_instance101/1(stop_out) -> t4/101
  mandelbroot_array_instance102/1(stop_out) -> t4/102
  mandelbroot_array_instance103/1(stop_out) -> t4/103
  mandelbroot_array_instance104/1(stop_out) -> t4/104
  mandelbroot_array_instance105/1(stop_out) -> t4/105
  mandelbroot_array_instance106/1(stop_out) -> t4/106
  mandelbroot_array_instance107/1(stop_out) -> t4/107
  mandelbroot_array_instance108/1(stop_out) -> t4/108
  mandelbroot_array_instance109/1(stop_out) -> t4/109
  mandelbroot_array_instance110/1(stop_out) -> t4/110
  mandelbroot_array_instance111/1(stop_out) -> t4/111
  mandelbroot_array_instance112/1(stop_out) -> t4/112
  mandelbroot_array_instance113/1(stop_out) -> t4/113
  mandelbroot_array_instance114/1(stop_out) -> t4/114
  mandelbroot_array_instance115/1(stop_out) -> t4/115
  mandelbroot_array_instance116/1(stop_out) -> t4/116
  mandelbroot_array_instance117/1(stop_out) -> t4/117
  mandelbroot_array_instance118/1(stop_out) -> t4/118
  mandelbroot_array_instance119/1(stop_out) -> t4/119
  mandelbroot_array_instance120/1(stop_out) -> t4/120
  mandelbroot_array_instance121/1(stop_out) -> t4/121
  mandelbroot_array_instance122/1(stop_out) -> t4/122
  mandelbroot_array_instance123/1(stop_out) -> t4/123
  mandelbroot_array_instance124/1(stop_out) -> t4/124
  mandelbroot_array_instance125/1(stop_out) -> t4/125
  mandelbroot_array_instance126/1(stop_out) -> t4/126
  mandelbroot_array_instance127/1(stop_out) -> t4/127
  mandelbroot_array_instance128/1(stop_out) -> t4/128
  t6/1 -> t7/1
  mandelbroot_array_instance1/2(z_out) -> t6/1
  mandelbroot_array_instance2/2(z_out) -> t6/2
  mandelbroot_array_instance3/2(z_out) -> t6/3
  mandelbroot_array_instance4/2(z_out) -> t6/4
  mandelbroot_array_instance5/2(z_out) -> t6/5
  mandelbroot_array_instance6/2(z_out) -> t6/6
  mandelbroot_array_instance7/2(z_out) -> t6/7
  mandelbroot_array_instance8/2(z_out) -> t6/8
  mandelbroot_array_instance9/2(z_out) -> t6/9
  mandelbroot_array_instance10/2(z_out) -> t6/10
  mandelbroot_array_instance11/2(z_out) -> t6/11
  mandelbroot_array_instance12/2(z_out) -> t6/12
  mandelbroot_array_instance13/2(z_out) -> t6/13
  mandelbroot_array_instance14/2(z_out) -> t6/14
  mandelbroot_array_instance15/2(z_out) -> t6/15
  mandelbroot_array_instance16/2(z_out) -> t6/16
  mandelbroot_array_instance17/2(z_out) -> t6/17
  mandelbroot_array_instance18/2(z_out) -> t6/18
  mandelbroot_array_instance19/2(z_out) -> t6/19
  mandelbroot_array_instance20/2(z_out) -> t6/20
  mandelbroot_array_instance21/2(z_out) -> t6/21
  mandelbroot_array_instance22/2(z_out) -> t6/22
  mandelbroot_array_instance23/2(z_out) -> t6/23
  mandelbroot_array_instance24/2(z_out) -> t6/24
  mandelbroot_array_instance25/2(z_out) -> t6/25
  mandelbroot_array_instance26/2(z_out) -> t6/26
  mandelbroot_array_instance27/2(z_out) -> t6/27
  mandelbroot_array_instance28/2(z_out) -> t6/28
  mandelbroot_array_instance29/2(z_out) -> t6/29
  mandelbroot_array_instance30/2(z_out) -> t6/30
  mandelbroot_array_instance31/2(z_out) -> t6/31
  mandelbroot_array_instance32/2(z_out) -> t6/32
  mandelbroot_array_instance33/2(z_out) -> t6/33
  mandelbroot_array_instance34/2(z_out) -> t6/34
  mandelbroot_array_instance35/2(z_out) -> t6/35
  mandelbroot_array_instance36/2(z_out) -> t6/36
  mandelbroot_array_instance37/2(z_out) -> t6/37
  mandelbroot_array_instance38/2(z_out) -> t6/38
  mandelbroot_array_instance39/2(z_out) -> t6/39
  mandelbroot_array_instance40/2(z_out) -> t6/40
  mandelbroot_array_instance41/2(z_out) -> t6/41
  mandelbroot_array_instance42/2(z_out) -> t6/42
  mandelbroot_array_instance43/2(z_out) -> t6/43
  mandelbroot_array_instance44/2(z_out) -> t6/44
  mandelbroot_array_instance45/2(z_out) -> t6/45
  mandelbroot_array_instance46/2(z_out) -> t6/46
  mandelbroot_array_instance47/2(z_out) -> t6/47
  mandelbroot_array_instance48/2(z_out) -> t6/48
  mandelbroot_array_instance49/2(z_out) -> t6/49
  mandelbroot_array_instance50/2(z_out) -> t6/50
  mandelbroot_array_instance51/2(z_out) -> t6/51
  mandelbroot_array_instance52/2(z_out) -> t6/52
  mandelbroot_array_instance53/2(z_out) -> t6/53
  mandelbroot_array_instance54/2(z_out) -> t6/54
  mandelbroot_array_instance55/2(z_out) -> t6/55
  mandelbroot_array_instance56/2(z_out) -> t6/56
  mandelbroot_array_instance57/2(z_out) -> t6/57
  mandelbroot_array_instance58/2(z_out) -> t6/58
  mandelbroot_array_instance59/2(z_out) -> t6/59
  mandelbroot_array_instance60/2(z_out) -> t6/60
  mandelbroot_array_instance61/2(z_out) -> t6/61
  mandelbroot_array_instance62/2(z_out) -> t6/62
  mandelbroot_array_instance63/2(z_out) -> t6/63
  mandelbroot_array_instance64/2(z_out) -> t6/64
  mandelbroot_array_instance65/2(z_out) -> t6/65
  mandelbroot_array_instance66/2(z_out) -> t6/66
  mandelbroot_array_instance67/2(z_out) -> t6/67
  mandelbroot_array_instance68/2(z_out) -> t6/68
  mandelbroot_array_instance69/2(z_out) -> t6/69
  mandelbroot_array_instance70/2(z_out) -> t6/70
  mandelbroot_array_instance71/2(z_out) -> t6/71
  mandelbroot_array_instance72/2(z_out) -> t6/72
  mandelbroot_array_instance73/2(z_out) -> t6/73
  mandelbroot_array_instance74/2(z_out) -> t6/74
  mandelbroot_array_instance75/2(z_out) -> t6/75
  mandelbroot_array_instance76/2(z_out) -> t6/76
  mandelbroot_array_instance77/2(z_out) -> t6/77
  mandelbroot_array_instance78/2(z_out) -> t6/78
  mandelbroot_array_instance79/2(z_out) -> t6/79
  mandelbroot_array_instance80/2(z_out) -> t6/80
  mandelbroot_array_instance81/2(z_out) -> t6/81
  mandelbroot_array_instance82/2(z_out) -> t6/82
  mandelbroot_array_instance83/2(z_out) -> t6/83
  mandelbroot_array_instance84/2(z_out) -> t6/84
  mandelbroot_array_instance85/2(z_out) -> t6/85
  mandelbroot_array_instance86/2(z_out) -> t6/86
  mandelbroot_array_instance87/2(z_out) -> t6/87
  mandelbroot_array_instance88/2(z_out) -> t6/88
  mandelbroot_array_instance89/2(z_out) -> t6/89
  mandelbroot_array_instance90/2(z_out) -> t6/90
  mandelbroot_array_instance91/2(z_out) -> t6/91
  mandelbroot_array_instance92/2(z_out) -> t6/92
  mandelbroot_array_instance93/2(z_out) -> t6/93
  mandelbroot_array_instance94/2(z_out) -> t6/94
  mandelbroot_array_instance95/2(z_out) -> t6/95
  mandelbroot_array_instance96/2(z_out) -> t6/96
  mandelbroot_array_instance97/2(z_out) -> t6/97
  mandelbroot_array_instance98/2(z_out) -> t6/98
  mandelbroot_array_instance99/2(z_out) -> t6/99
  mandelbroot_array_instance100/2(z_out) -> t6/100
  mandelbroot_array_instance101/2(z_out) -> t6/101
  mandelbroot_array_instance102/2(z_out) -> t6/102
  mandelbroot_array_instance103/2(z_out) -> t6/103
  mandelbroot_array_instance104/2(z_out) -> t6/104
  mandelbroot_array_instance105/2(z_out) -> t6/105
  mandelbroot_array_instance106/2(z_out) -> t6/106
  mandelbroot_array_instance107/2(z_out) -> t6/107
  mandelbroot_array_instance108/2(z_out) -> t6/108
  mandelbroot_array_instance109/2(z_out) -> t6/109
  mandelbroot_array_instance110/2(z_out) -> t6/110
  mandelbroot_array_instance111/2(z_out) -> t6/111
  mandelbroot_array_instance112/2(z_out) -> t6/112
  mandelbroot_array_instance113/2(z_out) -> t6/113
  mandelbroot_array_instance114/2(z_out) -> t6/114
  mandelbroot_array_instance115/2(z_out) -> t6/115
  mandelbroot_array_instance116/2(z_out) -> t6/116
  mandelbroot_array_instance117/2(z_out) -> t6/117
  mandelbroot_array_instance118/2(z_out) -> t6/118
  mandelbroot_array_instance119/2(z_out) -> t6/119
  mandelbroot_array_instance120/2(z_out) -> t6/120
  mandelbroot_array_instance121/2(z_out) -> t6/121
  mandelbroot_array_instance122/2(z_out) -> t6/122
  mandelbroot_array_instance123/2(z_out) -> t6/123
  mandelbroot_array_instance124/2(z_out) -> t6/124
  mandelbroot_array_instance125/2(z_out) -> t6/125
  mandelbroot_array_instance126/2(z_out) -> t6/126
  mandelbroot_array_instance127/2(z_out) -> t6/127
  mandelbroot_array_instance128/2(z_out) -> t6/128
  t8/1 -> t9/1
  mandelbroot_array_instance1/3(c_out) -> t8/1
  mandelbroot_array_instance2/3(c_out) -> t8/2
  mandelbroot_array_instance3/3(c_out) -> t8/3
  mandelbroot_array_instance4/3(c_out) -> t8/4
  mandelbroot_array_instance5/3(c_out) -> t8/5
  mandelbroot_array_instance6/3(c_out) -> t8/6
  mandelbroot_array_instance7/3(c_out) -> t8/7
  mandelbroot_array_instance8/3(c_out) -> t8/8
  mandelbroot_array_instance9/3(c_out) -> t8/9
  mandelbroot_array_instance10/3(c_out) -> t8/10
  mandelbroot_array_instance11/3(c_out) -> t8/11
  mandelbroot_array_instance12/3(c_out) -> t8/12
  mandelbroot_array_instance13/3(c_out) -> t8/13
  mandelbroot_array_instance14/3(c_out) -> t8/14
  mandelbroot_array_instance15/3(c_out) -> t8/15
  mandelbroot_array_instance16/3(c_out) -> t8/16
  mandelbroot_array_instance17/3(c_out) -> t8/17
  mandelbroot_array_instance18/3(c_out) -> t8/18
  mandelbroot_array_instance19/3(c_out) -> t8/19
  mandelbroot_array_instance20/3(c_out) -> t8/20
  mandelbroot_array_instance21/3(c_out) -> t8/21
  mandelbroot_array_instance22/3(c_out) -> t8/22
  mandelbroot_array_instance23/3(c_out) -> t8/23
  mandelbroot_array_instance24/3(c_out) -> t8/24
  mandelbroot_array_instance25/3(c_out) -> t8/25
  mandelbroot_array_instance26/3(c_out) -> t8/26
  mandelbroot_array_instance27/3(c_out) -> t8/27
  mandelbroot_array_instance28/3(c_out) -> t8/28
  mandelbroot_array_instance29/3(c_out) -> t8/29
  mandelbroot_array_instance30/3(c_out) -> t8/30
  mandelbroot_array_instance31/3(c_out) -> t8/31
  mandelbroot_array_instance32/3(c_out) -> t8/32
  mandelbroot_array_instance33/3(c_out) -> t8/33
  mandelbroot_array_instance34/3(c_out) -> t8/34
  mandelbroot_array_instance35/3(c_out) -> t8/35
  mandelbroot_array_instance36/3(c_out) -> t8/36
  mandelbroot_array_instance37/3(c_out) -> t8/37
  mandelbroot_array_instance38/3(c_out) -> t8/38
  mandelbroot_array_instance39/3(c_out) -> t8/39
  mandelbroot_array_instance40/3(c_out) -> t8/40
  mandelbroot_array_instance41/3(c_out) -> t8/41
  mandelbroot_array_instance42/3(c_out) -> t8/42
  mandelbroot_array_instance43/3(c_out) -> t8/43
  mandelbroot_array_instance44/3(c_out) -> t8/44
  mandelbroot_array_instance45/3(c_out) -> t8/45
  mandelbroot_array_instance46/3(c_out) -> t8/46
  mandelbroot_array_instance47/3(c_out) -> t8/47
  mandelbroot_array_instance48/3(c_out) -> t8/48
  mandelbroot_array_instance49/3(c_out) -> t8/49
  mandelbroot_array_instance50/3(c_out) -> t8/50
  mandelbroot_array_instance51/3(c_out) -> t8/51
  mandelbroot_array_instance52/3(c_out) -> t8/52
  mandelbroot_array_instance53/3(c_out) -> t8/53
  mandelbroot_array_instance54/3(c_out) -> t8/54
  mandelbroot_array_instance55/3(c_out) -> t8/55
  mandelbroot_array_instance56/3(c_out) -> t8/56
  mandelbroot_array_instance57/3(c_out) -> t8/57
  mandelbroot_array_instance58/3(c_out) -> t8/58
  mandelbroot_array_instance59/3(c_out) -> t8/59
  mandelbroot_array_instance60/3(c_out) -> t8/60
  mandelbroot_array_instance61/3(c_out) -> t8/61
  mandelbroot_array_instance62/3(c_out) -> t8/62
  mandelbroot_array_instance63/3(c_out) -> t8/63
  mandelbroot_array_instance64/3(c_out) -> t8/64
  mandelbroot_array_instance65/3(c_out) -> t8/65
  mandelbroot_array_instance66/3(c_out) -> t8/66
  mandelbroot_array_instance67/3(c_out) -> t8/67
  mandelbroot_array_instance68/3(c_out) -> t8/68
  mandelbroot_array_instance69/3(c_out) -> t8/69
  mandelbroot_array_instance70/3(c_out) -> t8/70
  mandelbroot_array_instance71/3(c_out) -> t8/71
  mandelbroot_array_instance72/3(c_out) -> t8/72
  mandelbroot_array_instance73/3(c_out) -> t8/73
  mandelbroot_array_instance74/3(c_out) -> t8/74
  mandelbroot_array_instance75/3(c_out) -> t8/75
  mandelbroot_array_instance76/3(c_out) -> t8/76
  mandelbroot_array_instance77/3(c_out) -> t8/77
  mandelbroot_array_instance78/3(c_out) -> t8/78
  mandelbroot_array_instance79/3(c_out) -> t8/79
  mandelbroot_array_instance80/3(c_out) -> t8/80
  mandelbroot_array_instance81/3(c_out) -> t8/81
  mandelbroot_array_instance82/3(c_out) -> t8/82
  mandelbroot_array_instance83/3(c_out) -> t8/83
  mandelbroot_array_instance84/3(c_out) -> t8/84
  mandelbroot_array_instance85/3(c_out) -> t8/85
  mandelbroot_array_instance86/3(c_out) -> t8/86
  mandelbroot_array_instance87/3(c_out) -> t8/87
  mandelbroot_array_instance88/3(c_out) -> t8/88
  mandelbroot_array_instance89/3(c_out) -> t8/89
  mandelbroot_array_instance90/3(c_out) -> t8/90
  mandelbroot_array_instance91/3(c_out) -> t8/91
  mandelbroot_array_instance92/3(c_out) -> t8/92
  mandelbroot_array_instance93/3(c_out) -> t8/93
  mandelbroot_array_instance94/3(c_out) -> t8/94
  mandelbroot_array_instance95/3(c_out) -> t8/95
  mandelbroot_array_instance96/3(c_out) -> t8/96
  mandelbroot_array_instance97/3(c_out) -> t8/97
  mandelbroot_array_instance98/3(c_out) -> t8/98
  mandelbroot_array_instance99/3(c_out) -> t8/99
  mandelbroot_array_instance100/3(c_out) -> t8/100
  mandelbroot_array_instance101/3(c_out) -> t8/101
  mandelbroot_array_instance102/3(c_out) -> t8/102
  mandelbroot_array_instance103/3(c_out) -> t8/103
  mandelbroot_array_instance104/3(c_out) -> t8/104
  mandelbroot_array_instance105/3(c_out) -> t8/105
  mandelbroot_array_instance106/3(c_out) -> t8/106
  mandelbroot_array_instance107/3(c_out) -> t8/107
  mandelbroot_array_instance108/3(c_out) -> t8/108
  mandelbroot_array_instance109/3(c_out) -> t8/109
  mandelbroot_array_instance110/3(c_out) -> t8/110
  mandelbroot_array_instance111/3(c_out) -> t8/111
  mandelbroot_array_instance112/3(c_out) -> t8/112
  mandelbroot_array_instance113/3(c_out) -> t8/113
  mandelbroot_array_instance114/3(c_out) -> t8/114
  mandelbroot_array_instance115/3(c_out) -> t8/115
  mandelbroot_array_instance116/3(c_out) -> t8/116
  mandelbroot_array_instance117/3(c_out) -> t8/117
  mandelbroot_array_instance118/3(c_out) -> t8/118
  mandelbroot_array_instance119/3(c_out) -> t8/119
  mandelbroot_array_instance120/3(c_out) -> t8/120
  mandelbroot_array_instance121/3(c_out) -> t8/121
  mandelbroot_array_instance122/3(c_out) -> t8/122
  mandelbroot_array_instance123/3(c_out) -> t8/123
  mandelbroot_array_instance124/3(c_out) -> t8/124
  mandelbroot_array_instance125/3(c_out) -> t8/125
  mandelbroot_array_instance126/3(c_out) -> t8/126
  mandelbroot_array_instance127/3(c_out) -> t8/127
  mandelbroot_array_instance128/3(c_out) -> t8/128
  t10/1 -> t11/1
  mandelbroot_array_instance1/4(i_out) -> t10/1
  mandelbroot_array_instance2/4(i_out) -> t10/2
  mandelbroot_array_instance3/4(i_out) -> t10/3
  mandelbroot_array_instance4/4(i_out) -> t10/4
  mandelbroot_array_instance5/4(i_out) -> t10/5
  mandelbroot_array_instance6/4(i_out) -> t10/6
  mandelbroot_array_instance7/4(i_out) -> t10/7
  mandelbroot_array_instance8/4(i_out) -> t10/8
  mandelbroot_array_instance9/4(i_out) -> t10/9
  mandelbroot_array_instance10/4(i_out) -> t10/10
  mandelbroot_array_instance11/4(i_out) -> t10/11
  mandelbroot_array_instance12/4(i_out) -> t10/12
  mandelbroot_array_instance13/4(i_out) -> t10/13
  mandelbroot_array_instance14/4(i_out) -> t10/14
  mandelbroot_array_instance15/4(i_out) -> t10/15
  mandelbroot_array_instance16/4(i_out) -> t10/16
  mandelbroot_array_instance17/4(i_out) -> t10/17
  mandelbroot_array_instance18/4(i_out) -> t10/18
  mandelbroot_array_instance19/4(i_out) -> t10/19
  mandelbroot_array_instance20/4(i_out) -> t10/20
  mandelbroot_array_instance21/4(i_out) -> t10/21
  mandelbroot_array_instance22/4(i_out) -> t10/22
  mandelbroot_array_instance23/4(i_out) -> t10/23
  mandelbroot_array_instance24/4(i_out) -> t10/24
  mandelbroot_array_instance25/4(i_out) -> t10/25
  mandelbroot_array_instance26/4(i_out) -> t10/26
  mandelbroot_array_instance27/4(i_out) -> t10/27
  mandelbroot_array_instance28/4(i_out) -> t10/28
  mandelbroot_array_instance29/4(i_out) -> t10/29
  mandelbroot_array_instance30/4(i_out) -> t10/30
  mandelbroot_array_instance31/4(i_out) -> t10/31
  mandelbroot_array_instance32/4(i_out) -> t10/32
  mandelbroot_array_instance33/4(i_out) -> t10/33
  mandelbroot_array_instance34/4(i_out) -> t10/34
  mandelbroot_array_instance35/4(i_out) -> t10/35
  mandelbroot_array_instance36/4(i_out) -> t10/36
  mandelbroot_array_instance37/4(i_out) -> t10/37
  mandelbroot_array_instance38/4(i_out) -> t10/38
  mandelbroot_array_instance39/4(i_out) -> t10/39
  mandelbroot_array_instance40/4(i_out) -> t10/40
  mandelbroot_array_instance41/4(i_out) -> t10/41
  mandelbroot_array_instance42/4(i_out) -> t10/42
  mandelbroot_array_instance43/4(i_out) -> t10/43
  mandelbroot_array_instance44/4(i_out) -> t10/44
  mandelbroot_array_instance45/4(i_out) -> t10/45
  mandelbroot_array_instance46/4(i_out) -> t10/46
  mandelbroot_array_instance47/4(i_out) -> t10/47
  mandelbroot_array_instance48/4(i_out) -> t10/48
  mandelbroot_array_instance49/4(i_out) -> t10/49
  mandelbroot_array_instance50/4(i_out) -> t10/50
  mandelbroot_array_instance51/4(i_out) -> t10/51
  mandelbroot_array_instance52/4(i_out) -> t10/52
  mandelbroot_array_instance53/4(i_out) -> t10/53
  mandelbroot_array_instance54/4(i_out) -> t10/54
  mandelbroot_array_instance55/4(i_out) -> t10/55
  mandelbroot_array_instance56/4(i_out) -> t10/56
  mandelbroot_array_instance57/4(i_out) -> t10/57
  mandelbroot_array_instance58/4(i_out) -> t10/58
  mandelbroot_array_instance59/4(i_out) -> t10/59
  mandelbroot_array_instance60/4(i_out) -> t10/60
  mandelbroot_array_instance61/4(i_out) -> t10/61
  mandelbroot_array_instance62/4(i_out) -> t10/62
  mandelbroot_array_instance63/4(i_out) -> t10/63
  mandelbroot_array_instance64/4(i_out) -> t10/64
  mandelbroot_array_instance65/4(i_out) -> t10/65
  mandelbroot_array_instance66/4(i_out) -> t10/66
  mandelbroot_array_instance67/4(i_out) -> t10/67
  mandelbroot_array_instance68/4(i_out) -> t10/68
  mandelbroot_array_instance69/4(i_out) -> t10/69
  mandelbroot_array_instance70/4(i_out) -> t10/70
  mandelbroot_array_instance71/4(i_out) -> t10/71
  mandelbroot_array_instance72/4(i_out) -> t10/72
  mandelbroot_array_instance73/4(i_out) -> t10/73
  mandelbroot_array_instance74/4(i_out) -> t10/74
  mandelbroot_array_instance75/4(i_out) -> t10/75
  mandelbroot_array_instance76/4(i_out) -> t10/76
  mandelbroot_array_instance77/4(i_out) -> t10/77
  mandelbroot_array_instance78/4(i_out) -> t10/78
  mandelbroot_array_instance79/4(i_out) -> t10/79
  mandelbroot_array_instance80/4(i_out) -> t10/80
  mandelbroot_array_instance81/4(i_out) -> t10/81
  mandelbroot_array_instance82/4(i_out) -> t10/82
  mandelbroot_array_instance83/4(i_out) -> t10/83
  mandelbroot_array_instance84/4(i_out) -> t10/84
  mandelbroot_array_instance85/4(i_out) -> t10/85
  mandelbroot_array_instance86/4(i_out) -> t10/86
  mandelbroot_array_instance87/4(i_out) -> t10/87
  mandelbroot_array_instance88/4(i_out) -> t10/88
  mandelbroot_array_instance89/4(i_out) -> t10/89
  mandelbroot_array_instance90/4(i_out) -> t10/90
  mandelbroot_array_instance91/4(i_out) -> t10/91
  mandelbroot_array_instance92/4(i_out) -> t10/92
  mandelbroot_array_instance93/4(i_out) -> t10/93
  mandelbroot_array_instance94/4(i_out) -> t10/94
  mandelbroot_array_instance95/4(i_out) -> t10/95
  mandelbroot_array_instance96/4(i_out) -> t10/96
  mandelbroot_array_instance97/4(i_out) -> t10/97
  mandelbroot_array_instance98/4(i_out) -> t10/98
  mandelbroot_array_instance99/4(i_out) -> t10/99
  mandelbroot_array_instance100/4(i_out) -> t10/100
  mandelbroot_array_instance101/4(i_out) -> t10/101
  mandelbroot_array_instance102/4(i_out) -> t10/102
  mandelbroot_array_instance103/4(i_out) -> t10/103
  mandelbroot_array_instance104/4(i_out) -> t10/104
  mandelbroot_array_instance105/4(i_out) -> t10/105
  mandelbroot_array_instance106/4(i_out) -> t10/106
  mandelbroot_array_instance107/4(i_out) -> t10/107
  mandelbroot_array_instance108/4(i_out) -> t10/108
  mandelbroot_array_instance109/4(i_out) -> t10/109
  mandelbroot_array_instance110/4(i_out) -> t10/110
  mandelbroot_array_instance111/4(i_out) -> t10/111
  mandelbroot_array_instance112/4(i_out) -> t10/112
  mandelbroot_array_instance113/4(i_out) -> t10/113
  mandelbroot_array_instance114/4(i_out) -> t10/114
  mandelbroot_array_instance115/4(i_out) -> t10/115
  mandelbroot_array_instance116/4(i_out) -> t10/116
  mandelbroot_array_instance117/4(i_out) -> t10/117
  mandelbroot_array_instance118/4(i_out) -> t10/118
  mandelbroot_array_instance119/4(i_out) -> t10/119
  mandelbroot_array_instance120/4(i_out) -> t10/120
  mandelbroot_array_instance121/4(i_out) -> t10/121
  mandelbroot_array_instance122/4(i_out) -> t10/122
  mandelbroot_array_instance123/4(i_out) -> t10/123
  mandelbroot_array_instance124/4(i_out) -> t10/124
  mandelbroot_array_instance125/4(i_out) -> t10/125
  mandelbroot_array_instance126/4(i_out) -> t10/126
  mandelbroot_array_instance127/4(i_out) -> t10/127
  mandelbroot_array_instance128/4(i_out) -> t10/128
  t12/1 -> Demux_mux_1/1
  t12/2 -> Demux_mux_1/2
  t12/3 -> Demux_mux_1/3
  t12/4 -> Demux_mux_1/4
  t12/5 -> Demux_mux_1/5
  t12/6 -> Demux_mux_1/6
  t12/7 -> Demux_mux_1/7
  t12/8 -> Demux_mux_1/8
  t12/9 -> Demux_mux_1/9
  t12/10 -> Demux_mux_1/10
  t12/11 -> Demux_mux_1/11
  t12/12 -> Demux_mux_1/12
  t12/13 -> Demux_mux_1/13
  t12/14 -> Demux_mux_1/14
  t12/15 -> Demux_mux_1/15
  t12/16 -> Demux_mux_1/16
  t12/17 -> Demux_mux_1/17
  t12/18 -> Demux_mux_1/18
  t12/19 -> Demux_mux_1/19
  t12/20 -> Demux_mux_1/20
  t12/21 -> Demux_mux_1/21
  t12/22 -> Demux_mux_1/22
  t12/23 -> Demux_mux_1/23
  t12/24 -> Demux_mux_1/24
  t12/25 -> Demux_mux_1/25
  t12/26 -> Demux_mux_1/26
  t12/27 -> Demux_mux_1/27
  t12/28 -> Demux_mux_1/28
  t12/29 -> Demux_mux_1/29
  t12/30 -> Demux_mux_1/30
  t12/31 -> Demux_mux_1/31
  t12/32 -> Demux_mux_1/32
  t12/33 -> Demux_mux_1/33
  t12/34 -> Demux_mux_1/34
  t12/35 -> Demux_mux_1/35
  t12/36 -> Demux_mux_1/36
  t12/37 -> Demux_mux_1/37
  t12/38 -> Demux_mux_1/38
  t12/39 -> Demux_mux_1/39
  t12/40 -> Demux_mux_1/40
  t12/41 -> Demux_mux_1/41
  t12/42 -> Demux_mux_1/42
  t12/43 -> Demux_mux_1/43
  t12/44 -> Demux_mux_1/44
  t12/45 -> Demux_mux_1/45
  t12/46 -> Demux_mux_1/46
  t12/47 -> Demux_mux_1/47
  t12/48 -> Demux_mux_1/48
  t12/49 -> Demux_mux_1/49
  t12/50 -> Demux_mux_1/50
  t12/51 -> Demux_mux_1/51
  t12/52 -> Demux_mux_1/52
  t12/53 -> Demux_mux_1/53
  t12/54 -> Demux_mux_1/54
  t12/55 -> Demux_mux_1/55
  t12/56 -> Demux_mux_1/56
  t12/57 -> Demux_mux_1/57
  t12/58 -> Demux_mux_1/58
  t12/59 -> Demux_mux_1/59
  t12/60 -> Demux_mux_1/60
  t12/61 -> Demux_mux_1/61
  t12/62 -> Demux_mux_1/62
  t12/63 -> Demux_mux_1/63
  t12/64 -> Demux_mux_1/64
  t12/65 -> Demux_mux_1/65
  t12/66 -> Demux_mux_1/66
  t12/67 -> Demux_mux_1/67
  t12/68 -> Demux_mux_1/68
  t12/69 -> Demux_mux_1/69
  t12/70 -> Demux_mux_1/70
  t12/71 -> Demux_mux_1/71
  t12/72 -> Demux_mux_1/72
  t12/73 -> Demux_mux_1/73
  t12/74 -> Demux_mux_1/74
  t12/75 -> Demux_mux_1/75
  t12/76 -> Demux_mux_1/76
  t12/77 -> Demux_mux_1/77
  t12/78 -> Demux_mux_1/78
  t12/79 -> Demux_mux_1/79
  t12/80 -> Demux_mux_1/80
  t12/81 -> Demux_mux_1/81
  t12/82 -> Demux_mux_1/82
  t12/83 -> Demux_mux_1/83
  t12/84 -> Demux_mux_1/84
  t12/85 -> Demux_mux_1/85
  t12/86 -> Demux_mux_1/86
  t12/87 -> Demux_mux_1/87
  t12/88 -> Demux_mux_1/88
  t12/89 -> Demux_mux_1/89
  t12/90 -> Demux_mux_1/90
  t12/91 -> Demux_mux_1/91
  t12/92 -> Demux_mux_1/92
  t12/93 -> Demux_mux_1/93
  t12/94 -> Demux_mux_1/94
  t12/95 -> Demux_mux_1/95
  t12/96 -> Demux_mux_1/96
  t12/97 -> Demux_mux_1/97
  t12/98 -> Demux_mux_1/98
  t12/99 -> Demux_mux_1/99
  t12/100 -> Demux_mux_1/100
  t12/101 -> Demux_mux_1/101
  t12/102 -> Demux_mux_1/102
  t12/103 -> Demux_mux_1/103
  t12/104 -> Demux_mux_1/104
  t12/105 -> Demux_mux_1/105
  t12/106 -> Demux_mux_1/106
  t12/107 -> Demux_mux_1/107
  t12/108 -> Demux_mux_1/108
  t12/109 -> Demux_mux_1/109
  t12/110 -> Demux_mux_1/110
  t12/111 -> Demux_mux_1/111
  t12/112 -> Demux_mux_1/112
  t12/113 -> Demux_mux_1/113
  t12/114 -> Demux_mux_1/114
  t12/115 -> Demux_mux_1/115
  t12/116 -> Demux_mux_1/116
  t12/117 -> Demux_mux_1/117
  t12/118 -> Demux_mux_1/118
  t12/119 -> Demux_mux_1/119
  t12/120 -> Demux_mux_1/120
  t12/121 -> Demux_mux_1/121
  t12/122 -> Demux_mux_1/122
  t12/123 -> Demux_mux_1/123
  t12/124 -> Demux_mux_1/124
  t12/125 -> Demux_mux_1/125
  t12/126 -> Demux_mux_1/126
  t12/127 -> Demux_mux_1/127
  t12/128 -> Terminator2/1
  t13/1 -> Demux1_mux_1/1
  t13/2 -> Demux1_mux_1/2
  t13/3 -> Demux1_mux_1/3
  t13/4 -> Demux1_mux_1/4
  t13/5 -> Demux1_mux_1/5
  t13/6 -> Demux1_mux_1/6
  t13/7 -> Demux1_mux_1/7
  t13/8 -> Demux1_mux_1/8
  t13/9 -> Demux1_mux_1/9
  t13/10 -> Demux1_mux_1/10
  t13/11 -> Demux1_mux_1/11
  t13/12 -> Demux1_mux_1/12
  t13/13 -> Demux1_mux_1/13
  t13/14 -> Demux1_mux_1/14
  t13/15 -> Demux1_mux_1/15
  t13/16 -> Demux1_mux_1/16
  t13/17 -> Demux1_mux_1/17
  t13/18 -> Demux1_mux_1/18
  t13/19 -> Demux1_mux_1/19
  t13/20 -> Demux1_mux_1/20
  t13/21 -> Demux1_mux_1/21
  t13/22 -> Demux1_mux_1/22
  t13/23 -> Demux1_mux_1/23
  t13/24 -> Demux1_mux_1/24
  t13/25 -> Demux1_mux_1/25
  t13/26 -> Demux1_mux_1/26
  t13/27 -> Demux1_mux_1/27
  t13/28 -> Demux1_mux_1/28
  t13/29 -> Demux1_mux_1/29
  t13/30 -> Demux1_mux_1/30
  t13/31 -> Demux1_mux_1/31
  t13/32 -> Demux1_mux_1/32
  t13/33 -> Demux1_mux_1/33
  t13/34 -> Demux1_mux_1/34
  t13/35 -> Demux1_mux_1/35
  t13/36 -> Demux1_mux_1/36
  t13/37 -> Demux1_mux_1/37
  t13/38 -> Demux1_mux_1/38
  t13/39 -> Demux1_mux_1/39
  t13/40 -> Demux1_mux_1/40
  t13/41 -> Demux1_mux_1/41
  t13/42 -> Demux1_mux_1/42
  t13/43 -> Demux1_mux_1/43
  t13/44 -> Demux1_mux_1/44
  t13/45 -> Demux1_mux_1/45
  t13/46 -> Demux1_mux_1/46
  t13/47 -> Demux1_mux_1/47
  t13/48 -> Demux1_mux_1/48
  t13/49 -> Demux1_mux_1/49
  t13/50 -> Demux1_mux_1/50
  t13/51 -> Demux1_mux_1/51
  t13/52 -> Demux1_mux_1/52
  t13/53 -> Demux1_mux_1/53
  t13/54 -> Demux1_mux_1/54
  t13/55 -> Demux1_mux_1/55
  t13/56 -> Demux1_mux_1/56
  t13/57 -> Demux1_mux_1/57
  t13/58 -> Demux1_mux_1/58
  t13/59 -> Demux1_mux_1/59
  t13/60 -> Demux1_mux_1/60
  t13/61 -> Demux1_mux_1/61
  t13/62 -> Demux1_mux_1/62
  t13/63 -> Demux1_mux_1/63
  t13/64 -> Demux1_mux_1/64
  t13/65 -> Demux1_mux_1/65
  t13/66 -> Demux1_mux_1/66
  t13/67 -> Demux1_mux_1/67
  t13/68 -> Demux1_mux_1/68
  t13/69 -> Demux1_mux_1/69
  t13/70 -> Demux1_mux_1/70
  t13/71 -> Demux1_mux_1/71
  t13/72 -> Demux1_mux_1/72
  t13/73 -> Demux1_mux_1/73
  t13/74 -> Demux1_mux_1/74
  t13/75 -> Demux1_mux_1/75
  t13/76 -> Demux1_mux_1/76
  t13/77 -> Demux1_mux_1/77
  t13/78 -> Demux1_mux_1/78
  t13/79 -> Demux1_mux_1/79
  t13/80 -> Demux1_mux_1/80
  t13/81 -> Demux1_mux_1/81
  t13/82 -> Demux1_mux_1/82
  t13/83 -> Demux1_mux_1/83
  t13/84 -> Demux1_mux_1/84
  t13/85 -> Demux1_mux_1/85
  t13/86 -> Demux1_mux_1/86
  t13/87 -> Demux1_mux_1/87
  t13/88 -> Demux1_mux_1/88
  t13/89 -> Demux1_mux_1/89
  t13/90 -> Demux1_mux_1/90
  t13/91 -> Demux1_mux_1/91
  t13/92 -> Demux1_mux_1/92
  t13/93 -> Demux1_mux_1/93
  t13/94 -> Demux1_mux_1/94
  t13/95 -> Demux1_mux_1/95
  t13/96 -> Demux1_mux_1/96
  t13/97 -> Demux1_mux_1/97
  t13/98 -> Demux1_mux_1/98
  t13/99 -> Demux1_mux_1/99
  t13/100 -> Demux1_mux_1/100
  t13/101 -> Demux1_mux_1/101
  t13/102 -> Demux1_mux_1/102
  t13/103 -> Demux1_mux_1/103
  t13/104 -> Demux1_mux_1/104
  t13/105 -> Demux1_mux_1/105
  t13/106 -> Demux1_mux_1/106
  t13/107 -> Demux1_mux_1/107
  t13/108 -> Demux1_mux_1/108
  t13/109 -> Demux1_mux_1/109
  t13/110 -> Demux1_mux_1/110
  t13/111 -> Demux1_mux_1/111
  t13/112 -> Demux1_mux_1/112
  t13/113 -> Demux1_mux_1/113
  t13/114 -> Demux1_mux_1/114
  t13/115 -> Demux1_mux_1/115
  t13/116 -> Demux1_mux_1/116
  t13/117 -> Demux1_mux_1/117
  t13/118 -> Demux1_mux_1/118
  t13/119 -> Demux1_mux_1/119
  t13/120 -> Demux1_mux_1/120
  t13/121 -> Demux1_mux_1/121
  t13/122 -> Demux1_mux_1/122
  t13/123 -> Demux1_mux_1/123
  t13/124 -> Demux1_mux_1/124
  t13/125 -> Demux1_mux_1/125
  t13/126 -> Demux1_mux_1/126
  t13/127 -> Demux1_mux_1/127
  t13/128 -> Terminator1/1
  t14/1 -> Demux2_mux_1/1
  t14/2 -> Demux2_mux_1/2
  t14/3 -> Demux2_mux_1/3
  t14/4 -> Demux2_mux_1/4
  t14/5 -> Demux2_mux_1/5
  t14/6 -> Demux2_mux_1/6
  t14/7 -> Demux2_mux_1/7
  t14/8 -> Demux2_mux_1/8
  t14/9 -> Demux2_mux_1/9
  t14/10 -> Demux2_mux_1/10
  t14/11 -> Demux2_mux_1/11
  t14/12 -> Demux2_mux_1/12
  t14/13 -> Demux2_mux_1/13
  t14/14 -> Demux2_mux_1/14
  t14/15 -> Demux2_mux_1/15
  t14/16 -> Demux2_mux_1/16
  t14/17 -> Demux2_mux_1/17
  t14/18 -> Demux2_mux_1/18
  t14/19 -> Demux2_mux_1/19
  t14/20 -> Demux2_mux_1/20
  t14/21 -> Demux2_mux_1/21
  t14/22 -> Demux2_mux_1/22
  t14/23 -> Demux2_mux_1/23
  t14/24 -> Demux2_mux_1/24
  t14/25 -> Demux2_mux_1/25
  t14/26 -> Demux2_mux_1/26
  t14/27 -> Demux2_mux_1/27
  t14/28 -> Demux2_mux_1/28
  t14/29 -> Demux2_mux_1/29
  t14/30 -> Demux2_mux_1/30
  t14/31 -> Demux2_mux_1/31
  t14/32 -> Demux2_mux_1/32
  t14/33 -> Demux2_mux_1/33
  t14/34 -> Demux2_mux_1/34
  t14/35 -> Demux2_mux_1/35
  t14/36 -> Demux2_mux_1/36
  t14/37 -> Demux2_mux_1/37
  t14/38 -> Demux2_mux_1/38
  t14/39 -> Demux2_mux_1/39
  t14/40 -> Demux2_mux_1/40
  t14/41 -> Demux2_mux_1/41
  t14/42 -> Demux2_mux_1/42
  t14/43 -> Demux2_mux_1/43
  t14/44 -> Demux2_mux_1/44
  t14/45 -> Demux2_mux_1/45
  t14/46 -> Demux2_mux_1/46
  t14/47 -> Demux2_mux_1/47
  t14/48 -> Demux2_mux_1/48
  t14/49 -> Demux2_mux_1/49
  t14/50 -> Demux2_mux_1/50
  t14/51 -> Demux2_mux_1/51
  t14/52 -> Demux2_mux_1/52
  t14/53 -> Demux2_mux_1/53
  t14/54 -> Demux2_mux_1/54
  t14/55 -> Demux2_mux_1/55
  t14/56 -> Demux2_mux_1/56
  t14/57 -> Demux2_mux_1/57
  t14/58 -> Demux2_mux_1/58
  t14/59 -> Demux2_mux_1/59
  t14/60 -> Demux2_mux_1/60
  t14/61 -> Demux2_mux_1/61
  t14/62 -> Demux2_mux_1/62
  t14/63 -> Demux2_mux_1/63
  t14/64 -> Demux2_mux_1/64
  t14/65 -> Demux2_mux_1/65
  t14/66 -> Demux2_mux_1/66
  t14/67 -> Demux2_mux_1/67
  t14/68 -> Demux2_mux_1/68
  t14/69 -> Demux2_mux_1/69
  t14/70 -> Demux2_mux_1/70
  t14/71 -> Demux2_mux_1/71
  t14/72 -> Demux2_mux_1/72
  t14/73 -> Demux2_mux_1/73
  t14/74 -> Demux2_mux_1/74
  t14/75 -> Demux2_mux_1/75
  t14/76 -> Demux2_mux_1/76
  t14/77 -> Demux2_mux_1/77
  t14/78 -> Demux2_mux_1/78
  t14/79 -> Demux2_mux_1/79
  t14/80 -> Demux2_mux_1/80
  t14/81 -> Demux2_mux_1/81
  t14/82 -> Demux2_mux_1/82
  t14/83 -> Demux2_mux_1/83
  t14/84 -> Demux2_mux_1/84
  t14/85 -> Demux2_mux_1/85
  t14/86 -> Demux2_mux_1/86
  t14/87 -> Demux2_mux_1/87
  t14/88 -> Demux2_mux_1/88
  t14/89 -> Demux2_mux_1/89
  t14/90 -> Demux2_mux_1/90
  t14/91 -> Demux2_mux_1/91
  t14/92 -> Demux2_mux_1/92
  t14/93 -> Demux2_mux_1/93
  t14/94 -> Demux2_mux_1/94
  t14/95 -> Demux2_mux_1/95
  t14/96 -> Demux2_mux_1/96
  t14/97 -> Demux2_mux_1/97
  t14/98 -> Demux2_mux_1/98
  t14/99 -> Demux2_mux_1/99
  t14/100 -> Demux2_mux_1/100
  t14/101 -> Demux2_mux_1/101
  t14/102 -> Demux2_mux_1/102
  t14/103 -> Demux2_mux_1/103
  t14/104 -> Demux2_mux_1/104
  t14/105 -> Demux2_mux_1/105
  t14/106 -> Demux2_mux_1/106
  t14/107 -> Demux2_mux_1/107
  t14/108 -> Demux2_mux_1/108
  t14/109 -> Demux2_mux_1/109
  t14/110 -> Demux2_mux_1/110
  t14/111 -> Demux2_mux_1/111
  t14/112 -> Demux2_mux_1/112
  t14/113 -> Demux2_mux_1/113
  t14/114 -> Demux2_mux_1/114
  t14/115 -> Demux2_mux_1/115
  t14/116 -> Demux2_mux_1/116
  t14/117 -> Demux2_mux_1/117
  t14/118 -> Demux2_mux_1/118
  t14/119 -> Demux2_mux_1/119
  t14/120 -> Demux2_mux_1/120
  t14/121 -> Demux2_mux_1/121
  t14/122 -> Demux2_mux_1/122
  t14/123 -> Demux2_mux_1/123
  t14/124 -> Demux2_mux_1/124
  t14/125 -> Demux2_mux_1/125
  t14/126 -> Demux2_mux_1/126
  t14/127 -> Demux2_mux_1/127
  t14/128 -> Terminator/1
  t15/1 -> Demux3_mux_1/1
  t15/2 -> Demux3_mux_1/2
  t15/3 -> Demux3_mux_1/3
  t15/4 -> Demux3_mux_1/4
  t15/5 -> Demux3_mux_1/5
  t15/6 -> Demux3_mux_1/6
  t15/7 -> Demux3_mux_1/7
  t15/8 -> Demux3_mux_1/8
  t15/9 -> Demux3_mux_1/9
  t15/10 -> Demux3_mux_1/10
  t15/11 -> Demux3_mux_1/11
  t15/12 -> Demux3_mux_1/12
  t15/13 -> Demux3_mux_1/13
  t15/14 -> Demux3_mux_1/14
  t15/15 -> Demux3_mux_1/15
  t15/16 -> Demux3_mux_1/16
  t15/17 -> Demux3_mux_1/17
  t15/18 -> Demux3_mux_1/18
  t15/19 -> Demux3_mux_1/19
  t15/20 -> Demux3_mux_1/20
  t15/21 -> Demux3_mux_1/21
  t15/22 -> Demux3_mux_1/22
  t15/23 -> Demux3_mux_1/23
  t15/24 -> Demux3_mux_1/24
  t15/25 -> Demux3_mux_1/25
  t15/26 -> Demux3_mux_1/26
  t15/27 -> Demux3_mux_1/27
  t15/28 -> Demux3_mux_1/28
  t15/29 -> Demux3_mux_1/29
  t15/30 -> Demux3_mux_1/30
  t15/31 -> Demux3_mux_1/31
  t15/32 -> Demux3_mux_1/32
  t15/33 -> Demux3_mux_1/33
  t15/34 -> Demux3_mux_1/34
  t15/35 -> Demux3_mux_1/35
  t15/36 -> Demux3_mux_1/36
  t15/37 -> Demux3_mux_1/37
  t15/38 -> Demux3_mux_1/38
  t15/39 -> Demux3_mux_1/39
  t15/40 -> Demux3_mux_1/40
  t15/41 -> Demux3_mux_1/41
  t15/42 -> Demux3_mux_1/42
  t15/43 -> Demux3_mux_1/43
  t15/44 -> Demux3_mux_1/44
  t15/45 -> Demux3_mux_1/45
  t15/46 -> Demux3_mux_1/46
  t15/47 -> Demux3_mux_1/47
  t15/48 -> Demux3_mux_1/48
  t15/49 -> Demux3_mux_1/49
  t15/50 -> Demux3_mux_1/50
  t15/51 -> Demux3_mux_1/51
  t15/52 -> Demux3_mux_1/52
  t15/53 -> Demux3_mux_1/53
  t15/54 -> Demux3_mux_1/54
  t15/55 -> Demux3_mux_1/55
  t15/56 -> Demux3_mux_1/56
  t15/57 -> Demux3_mux_1/57
  t15/58 -> Demux3_mux_1/58
  t15/59 -> Demux3_mux_1/59
  t15/60 -> Demux3_mux_1/60
  t15/61 -> Demux3_mux_1/61
  t15/62 -> Demux3_mux_1/62
  t15/63 -> Demux3_mux_1/63
  t15/64 -> Demux3_mux_1/64
  t15/65 -> Demux3_mux_1/65
  t15/66 -> Demux3_mux_1/66
  t15/67 -> Demux3_mux_1/67
  t15/68 -> Demux3_mux_1/68
  t15/69 -> Demux3_mux_1/69
  t15/70 -> Demux3_mux_1/70
  t15/71 -> Demux3_mux_1/71
  t15/72 -> Demux3_mux_1/72
  t15/73 -> Demux3_mux_1/73
  t15/74 -> Demux3_mux_1/74
  t15/75 -> Demux3_mux_1/75
  t15/76 -> Demux3_mux_1/76
  t15/77 -> Demux3_mux_1/77
  t15/78 -> Demux3_mux_1/78
  t15/79 -> Demux3_mux_1/79
  t15/80 -> Demux3_mux_1/80
  t15/81 -> Demux3_mux_1/81
  t15/82 -> Demux3_mux_1/82
  t15/83 -> Demux3_mux_1/83
  t15/84 -> Demux3_mux_1/84
  t15/85 -> Demux3_mux_1/85
  t15/86 -> Demux3_mux_1/86
  t15/87 -> Demux3_mux_1/87
  t15/88 -> Demux3_mux_1/88
  t15/89 -> Demux3_mux_1/89
  t15/90 -> Demux3_mux_1/90
  t15/91 -> Demux3_mux_1/91
  t15/92 -> Demux3_mux_1/92
  t15/93 -> Demux3_mux_1/93
  t15/94 -> Demux3_mux_1/94
  t15/95 -> Demux3_mux_1/95
  t15/96 -> Demux3_mux_1/96
  t15/97 -> Demux3_mux_1/97
  t15/98 -> Demux3_mux_1/98
  t15/99 -> Demux3_mux_1/99
  t15/100 -> Demux3_mux_1/100
  t15/101 -> Demux3_mux_1/101
  t15/102 -> Demux3_mux_1/102
  t15/103 -> Demux3_mux_1/103
  t15/104 -> Demux3_mux_1/104
  t15/105 -> Demux3_mux_1/105
  t15/106 -> Demux3_mux_1/106
  t15/107 -> Demux3_mux_1/107
  t15/108 -> Demux3_mux_1/108
  t15/109 -> Demux3_mux_1/109
  t15/110 -> Demux3_mux_1/110
  t15/111 -> Demux3_mux_1/111
  t15/112 -> Demux3_mux_1/112
  t15/113 -> Demux3_mux_1/113
  t15/114 -> Demux3_mux_1/114
  t15/115 -> Demux3_mux_1/115
  t15/116 -> Demux3_mux_1/116
  t15/117 -> Demux3_mux_1/117
  t15/118 -> Demux3_mux_1/118
  t15/119 -> Demux3_mux_1/119
  t15/120 -> Demux3_mux_1/120
  t15/121 -> Demux3_mux_1/121
  t15/122 -> Demux3_mux_1/122
  t15/123 -> Demux3_mux_1/123
  t15/124 -> Demux3_mux_1/124
  t15/125 -> Demux3_mux_1/125
  t15/126 -> Demux3_mux_1/126
  t15/127 -> Demux3_mux_1/127
  t15/128 -> result/1
  t16/1 -> concatenate/2
  t16/2 -> concatenate/3
  t16/3 -> concatenate/4
  t16/4 -> concatenate/5
  t16/5 -> concatenate/6
  t16/6 -> concatenate/7
  t16/7 -> concatenate/8
  t16/8 -> concatenate/9
  t16/9 -> concatenate/10
  t16/10 -> concatenate/11
  t16/11 -> concatenate/12
  t16/12 -> concatenate/13
  t16/13 -> concatenate/14
  t16/14 -> concatenate/15
  t16/15 -> concatenate/16
  t16/16 -> concatenate/17
  t16/17 -> concatenate/18
  t16/18 -> concatenate/19
  t16/19 -> concatenate/20
  t16/20 -> concatenate/21
  t16/21 -> concatenate/22
  t16/22 -> concatenate/23
  t16/23 -> concatenate/24
  t16/24 -> concatenate/25
  t16/25 -> concatenate/26
  t16/26 -> concatenate/27
  t16/27 -> concatenate/28
  t16/28 -> concatenate/29
  t16/29 -> concatenate/30
  t16/30 -> concatenate/31
  t16/31 -> concatenate/32
  t16/32 -> concatenate/33
  t16/33 -> concatenate/34
  t16/34 -> concatenate/35
  t16/35 -> concatenate/36
  t16/36 -> concatenate/37
  t16/37 -> concatenate/38
  t16/38 -> concatenate/39
  t16/39 -> concatenate/40
  t16/40 -> concatenate/41
  t16/41 -> concatenate/42
  t16/42 -> concatenate/43
  t16/43 -> concatenate/44
  t16/44 -> concatenate/45
  t16/45 -> concatenate/46
  t16/46 -> concatenate/47
  t16/47 -> concatenate/48
  t16/48 -> concatenate/49
  t16/49 -> concatenate/50
  t16/50 -> concatenate/51
  t16/51 -> concatenate/52
  t16/52 -> concatenate/53
  t16/53 -> concatenate/54
  t16/54 -> concatenate/55
  t16/55 -> concatenate/56
  t16/56 -> concatenate/57
  t16/57 -> concatenate/58
  t16/58 -> concatenate/59
  t16/59 -> concatenate/60
  t16/60 -> concatenate/61
  t16/61 -> concatenate/62
  t16/62 -> concatenate/63
  t16/63 -> concatenate/64
  t16/64 -> concatenate/65
  t16/65 -> concatenate/66
  t16/66 -> concatenate/67
  t16/67 -> concatenate/68
  t16/68 -> concatenate/69
  t16/69 -> concatenate/70
  t16/70 -> concatenate/71
  t16/71 -> concatenate/72
  t16/72 -> concatenate/73
  t16/73 -> concatenate/74
  t16/74 -> concatenate/75
  t16/75 -> concatenate/76
  t16/76 -> concatenate/77
  t16/77 -> concatenate/78
  t16/78 -> concatenate/79
  t16/79 -> concatenate/80
  t16/80 -> concatenate/81
  t16/81 -> concatenate/82
  t16/82 -> concatenate/83
  t16/83 -> concatenate/84
  t16/84 -> concatenate/85
  t16/85 -> concatenate/86
  t16/86 -> concatenate/87
  t16/87 -> concatenate/88
  t16/88 -> concatenate/89
  t16/89 -> concatenate/90
  t16/90 -> concatenate/91
  t16/91 -> concatenate/92
  t16/92 -> concatenate/93
  t16/93 -> concatenate/94
  t16/94 -> concatenate/95
  t16/95 -> concatenate/96
  t16/96 -> concatenate/97
  t16/97 -> concatenate/98
  t16/98 -> concatenate/99
  t16/99 -> concatenate/100
  t16/100 -> concatenate/101
  t16/101 -> concatenate/102
  t16/102 -> concatenate/103
  t16/103 -> concatenate/104
  t16/104 -> concatenate/105
  t16/105 -> concatenate/106
  t16/106 -> concatenate/107
  t16/107 -> concatenate/108
  t16/108 -> concatenate/109
  t16/109 -> concatenate/110
  t16/110 -> concatenate/111
  t16/111 -> concatenate/112
  t16/112 -> concatenate/113
  t16/113 -> concatenate/114
  t16/114 -> concatenate/115
  t16/115 -> concatenate/116
  t16/116 -> concatenate/117
  t16/117 -> concatenate/118
  t16/118 -> concatenate/119
  t16/119 -> concatenate/120
  t16/120 -> concatenate/121
  t16/121 -> concatenate/122
  t16/122 -> concatenate/123
  t16/123 -> concatenate/124
  t16/124 -> concatenate/125
  t16/125 -> concatenate/126
  t16/126 -> concatenate/127
  t16/127 -> concatenate/128
  t17/1 -> concatenate1/2
  t17/2 -> concatenate1/3
  t17/3 -> concatenate1/4
  t17/4 -> concatenate1/5
  t17/5 -> concatenate1/6
  t17/6 -> concatenate1/7
  t17/7 -> concatenate1/8
  t17/8 -> concatenate1/9
  t17/9 -> concatenate1/10
  t17/10 -> concatenate1/11
  t17/11 -> concatenate1/12
  t17/12 -> concatenate1/13
  t17/13 -> concatenate1/14
  t17/14 -> concatenate1/15
  t17/15 -> concatenate1/16
  t17/16 -> concatenate1/17
  t17/17 -> concatenate1/18
  t17/18 -> concatenate1/19
  t17/19 -> concatenate1/20
  t17/20 -> concatenate1/21
  t17/21 -> concatenate1/22
  t17/22 -> concatenate1/23
  t17/23 -> concatenate1/24
  t17/24 -> concatenate1/25
  t17/25 -> concatenate1/26
  t17/26 -> concatenate1/27
  t17/27 -> concatenate1/28
  t17/28 -> concatenate1/29
  t17/29 -> concatenate1/30
  t17/30 -> concatenate1/31
  t17/31 -> concatenate1/32
  t17/32 -> concatenate1/33
  t17/33 -> concatenate1/34
  t17/34 -> concatenate1/35
  t17/35 -> concatenate1/36
  t17/36 -> concatenate1/37
  t17/37 -> concatenate1/38
  t17/38 -> concatenate1/39
  t17/39 -> concatenate1/40
  t17/40 -> concatenate1/41
  t17/41 -> concatenate1/42
  t17/42 -> concatenate1/43
  t17/43 -> concatenate1/44
  t17/44 -> concatenate1/45
  t17/45 -> concatenate1/46
  t17/46 -> concatenate1/47
  t17/47 -> concatenate1/48
  t17/48 -> concatenate1/49
  t17/49 -> concatenate1/50
  t17/50 -> concatenate1/51
  t17/51 -> concatenate1/52
  t17/52 -> concatenate1/53
  t17/53 -> concatenate1/54
  t17/54 -> concatenate1/55
  t17/55 -> concatenate1/56
  t17/56 -> concatenate1/57
  t17/57 -> concatenate1/58
  t17/58 -> concatenate1/59
  t17/59 -> concatenate1/60
  t17/60 -> concatenate1/61
  t17/61 -> concatenate1/62
  t17/62 -> concatenate1/63
  t17/63 -> concatenate1/64
  t17/64 -> concatenate1/65
  t17/65 -> concatenate1/66
  t17/66 -> concatenate1/67
  t17/67 -> concatenate1/68
  t17/68 -> concatenate1/69
  t17/69 -> concatenate1/70
  t17/70 -> concatenate1/71
  t17/71 -> concatenate1/72
  t17/72 -> concatenate1/73
  t17/73 -> concatenate1/74
  t17/74 -> concatenate1/75
  t17/75 -> concatenate1/76
  t17/76 -> concatenate1/77
  t17/77 -> concatenate1/78
  t17/78 -> concatenate1/79
  t17/79 -> concatenate1/80
  t17/80 -> concatenate1/81
  t17/81 -> concatenate1/82
  t17/82 -> concatenate1/83
  t17/83 -> concatenate1/84
  t17/84 -> concatenate1/85
  t17/85 -> concatenate1/86
  t17/86 -> concatenate1/87
  t17/87 -> concatenate1/88
  t17/88 -> concatenate1/89
  t17/89 -> concatenate1/90
  t17/90 -> concatenate1/91
  t17/91 -> concatenate1/92
  t17/92 -> concatenate1/93
  t17/93 -> concatenate1/94
  t17/94 -> concatenate1/95
  t17/95 -> concatenate1/96
  t17/96 -> concatenate1/97
  t17/97 -> concatenate1/98
  t17/98 -> concatenate1/99
  t17/99 -> concatenate1/100
  t17/100 -> concatenate1/101
  t17/101 -> concatenate1/102
  t17/102 -> concatenate1/103
  t17/103 -> concatenate1/104
  t17/104 -> concatenate1/105
  t17/105 -> concatenate1/106
  t17/106 -> concatenate1/107
  t17/107 -> concatenate1/108
  t17/108 -> concatenate1/109
  t17/109 -> concatenate1/110
  t17/110 -> concatenate1/111
  t17/111 -> concatenate1/112
  t17/112 -> concatenate1/113
  t17/113 -> concatenate1/114
  t17/114 -> concatenate1/115
  t17/115 -> concatenate1/116
  t17/116 -> concatenate1/117
  t17/117 -> concatenate1/118
  t17/118 -> concatenate1/119
  t17/119 -> concatenate1/120
  t17/120 -> concatenate1/121
  t17/121 -> concatenate1/122
  t17/122 -> concatenate1/123
  t17/123 -> concatenate1/124
  t17/124 -> concatenate1/125
  t17/125 -> concatenate1/126
  t17/126 -> concatenate1/127
  t17/127 -> concatenate1/128
  t18/1 -> concatenate2/2
  t18/2 -> concatenate2/3
  t18/3 -> concatenate2/4
  t18/4 -> concatenate2/5
  t18/5 -> concatenate2/6
  t18/6 -> concatenate2/7
  t18/7 -> concatenate2/8
  t18/8 -> concatenate2/9
  t18/9 -> concatenate2/10
  t18/10 -> concatenate2/11
  t18/11 -> concatenate2/12
  t18/12 -> concatenate2/13
  t18/13 -> concatenate2/14
  t18/14 -> concatenate2/15
  t18/15 -> concatenate2/16
  t18/16 -> concatenate2/17
  t18/17 -> concatenate2/18
  t18/18 -> concatenate2/19
  t18/19 -> concatenate2/20
  t18/20 -> concatenate2/21
  t18/21 -> concatenate2/22
  t18/22 -> concatenate2/23
  t18/23 -> concatenate2/24
  t18/24 -> concatenate2/25
  t18/25 -> concatenate2/26
  t18/26 -> concatenate2/27
  t18/27 -> concatenate2/28
  t18/28 -> concatenate2/29
  t18/29 -> concatenate2/30
  t18/30 -> concatenate2/31
  t18/31 -> concatenate2/32
  t18/32 -> concatenate2/33
  t18/33 -> concatenate2/34
  t18/34 -> concatenate2/35
  t18/35 -> concatenate2/36
  t18/36 -> concatenate2/37
  t18/37 -> concatenate2/38
  t18/38 -> concatenate2/39
  t18/39 -> concatenate2/40
  t18/40 -> concatenate2/41
  t18/41 -> concatenate2/42
  t18/42 -> concatenate2/43
  t18/43 -> concatenate2/44
  t18/44 -> concatenate2/45
  t18/45 -> concatenate2/46
  t18/46 -> concatenate2/47
  t18/47 -> concatenate2/48
  t18/48 -> concatenate2/49
  t18/49 -> concatenate2/50
  t18/50 -> concatenate2/51
  t18/51 -> concatenate2/52
  t18/52 -> concatenate2/53
  t18/53 -> concatenate2/54
  t18/54 -> concatenate2/55
  t18/55 -> concatenate2/56
  t18/56 -> concatenate2/57
  t18/57 -> concatenate2/58
  t18/58 -> concatenate2/59
  t18/59 -> concatenate2/60
  t18/60 -> concatenate2/61
  t18/61 -> concatenate2/62
  t18/62 -> concatenate2/63
  t18/63 -> concatenate2/64
  t18/64 -> concatenate2/65
  t18/65 -> concatenate2/66
  t18/66 -> concatenate2/67
  t18/67 -> concatenate2/68
  t18/68 -> concatenate2/69
  t18/69 -> concatenate2/70
  t18/70 -> concatenate2/71
  t18/71 -> concatenate2/72
  t18/72 -> concatenate2/73
  t18/73 -> concatenate2/74
  t18/74 -> concatenate2/75
  t18/75 -> concatenate2/76
  t18/76 -> concatenate2/77
  t18/77 -> concatenate2/78
  t18/78 -> concatenate2/79
  t18/79 -> concatenate2/80
  t18/80 -> concatenate2/81
  t18/81 -> concatenate2/82
  t18/82 -> concatenate2/83
  t18/83 -> concatenate2/84
  t18/84 -> concatenate2/85
  t18/85 -> concatenate2/86
  t18/86 -> concatenate2/87
  t18/87 -> concatenate2/88
  t18/88 -> concatenate2/89
  t18/89 -> concatenate2/90
  t18/90 -> concatenate2/91
  t18/91 -> concatenate2/92
  t18/92 -> concatenate2/93
  t18/93 -> concatenate2/94
  t18/94 -> concatenate2/95
  t18/95 -> concatenate2/96
  t18/96 -> concatenate2/97
  t18/97 -> concatenate2/98
  t18/98 -> concatenate2/99
  t18/99 -> concatenate2/100
  t18/100 -> concatenate2/101
  t18/101 -> concatenate2/102
  t18/102 -> concatenate2/103
  t18/103 -> concatenate2/104
  t18/104 -> concatenate2/105
  t18/105 -> concatenate2/106
  t18/106 -> concatenate2/107
  t18/107 -> concatenate2/108
  t18/108 -> concatenate2/109
  t18/109 -> concatenate2/110
  t18/110 -> concatenate2/111
  t18/111 -> concatenate2/112
  t18/112 -> concatenate2/113
  t18/113 -> concatenate2/114
  t18/114 -> concatenate2/115
  t18/115 -> concatenate2/116
  t18/116 -> concatenate2/117
  t18/117 -> concatenate2/118
  t18/118 -> concatenate2/119
  t18/119 -> concatenate2/120
  t18/120 -> concatenate2/121
  t18/121 -> concatenate2/122
  t18/122 -> concatenate2/123
  t18/123 -> concatenate2/124
  t18/124 -> concatenate2/125
  t18/125 -> concatenate2/126
  t18/126 -> concatenate2/127
  t18/127 -> concatenate2/128
  t19/1 -> concatenate3/2
  t19/2 -> concatenate3/3
  t19/3 -> concatenate3/4
  t19/4 -> concatenate3/5
  t19/5 -> concatenate3/6
  t19/6 -> concatenate3/7
  t19/7 -> concatenate3/8
  t19/8 -> concatenate3/9
  t19/9 -> concatenate3/10
  t19/10 -> concatenate3/11
  t19/11 -> concatenate3/12
  t19/12 -> concatenate3/13
  t19/13 -> concatenate3/14
  t19/14 -> concatenate3/15
  t19/15 -> concatenate3/16
  t19/16 -> concatenate3/17
  t19/17 -> concatenate3/18
  t19/18 -> concatenate3/19
  t19/19 -> concatenate3/20
  t19/20 -> concatenate3/21
  t19/21 -> concatenate3/22
  t19/22 -> concatenate3/23
  t19/23 -> concatenate3/24
  t19/24 -> concatenate3/25
  t19/25 -> concatenate3/26
  t19/26 -> concatenate3/27
  t19/27 -> concatenate3/28
  t19/28 -> concatenate3/29
  t19/29 -> concatenate3/30
  t19/30 -> concatenate3/31
  t19/31 -> concatenate3/32
  t19/32 -> concatenate3/33
  t19/33 -> concatenate3/34
  t19/34 -> concatenate3/35
  t19/35 -> concatenate3/36
  t19/36 -> concatenate3/37
  t19/37 -> concatenate3/38
  t19/38 -> concatenate3/39
  t19/39 -> concatenate3/40
  t19/40 -> concatenate3/41
  t19/41 -> concatenate3/42
  t19/42 -> concatenate3/43
  t19/43 -> concatenate3/44
  t19/44 -> concatenate3/45
  t19/45 -> concatenate3/46
  t19/46 -> concatenate3/47
  t19/47 -> concatenate3/48
  t19/48 -> concatenate3/49
  t19/49 -> concatenate3/50
  t19/50 -> concatenate3/51
  t19/51 -> concatenate3/52
  t19/52 -> concatenate3/53
  t19/53 -> concatenate3/54
  t19/54 -> concatenate3/55
  t19/55 -> concatenate3/56
  t19/56 -> concatenate3/57
  t19/57 -> concatenate3/58
  t19/58 -> concatenate3/59
  t19/59 -> concatenate3/60
  t19/60 -> concatenate3/61
  t19/61 -> concatenate3/62
  t19/62 -> concatenate3/63
  t19/63 -> concatenate3/64
  t19/64 -> concatenate3/65
  t19/65 -> concatenate3/66
  t19/66 -> concatenate3/67
  t19/67 -> concatenate3/68
  t19/68 -> concatenate3/69
  t19/69 -> concatenate3/70
  t19/70 -> concatenate3/71
  t19/71 -> concatenate3/72
  t19/72 -> concatenate3/73
  t19/73 -> concatenate3/74
  t19/74 -> concatenate3/75
  t19/75 -> concatenate3/76
  t19/76 -> concatenate3/77
  t19/77 -> concatenate3/78
  t19/78 -> concatenate3/79
  t19/79 -> concatenate3/80
  t19/80 -> concatenate3/81
  t19/81 -> concatenate3/82
  t19/82 -> concatenate3/83
  t19/83 -> concatenate3/84
  t19/84 -> concatenate3/85
  t19/85 -> concatenate3/86
  t19/86 -> concatenate3/87
  t19/87 -> concatenate3/88
  t19/88 -> concatenate3/89
  t19/89 -> concatenate3/90
  t19/90 -> concatenate3/91
  t19/91 -> concatenate3/92
  t19/92 -> concatenate3/93
  t19/93 -> concatenate3/94
  t19/94 -> concatenate3/95
  t19/95 -> concatenate3/96
  t19/96 -> concatenate3/97
  t19/97 -> concatenate3/98
  t19/98 -> concatenate3/99
  t19/99 -> concatenate3/100
  t19/100 -> concatenate3/101
  t19/101 -> concatenate3/102
  t19/102 -> concatenate3/103
  t19/103 -> concatenate3/104
  t19/104 -> concatenate3/105
  t19/105 -> concatenate3/106
  t19/106 -> concatenate3/107
  t19/107 -> concatenate3/108
  t19/108 -> concatenate3/109
  t19/109 -> concatenate3/110
  t19/110 -> concatenate3/111
  t19/111 -> concatenate3/112
  t19/112 -> concatenate3/113
  t19/113 -> concatenate3/114
  t19/114 -> concatenate3/115
  t19/115 -> concatenate3/116
  t19/116 -> concatenate3/117
  t19/117 -> concatenate3/118
  t19/118 -> concatenate3/119
  t19/119 -> concatenate3/120
  t19/120 -> concatenate3/121
  t19/121 -> concatenate3/122
  t19/122 -> concatenate3/123
  t19/123 -> concatenate3/124
  t19/124 -> concatenate3/125
  t19/125 -> concatenate3/126
  t19/126 -> concatenate3/127
  t19/127 -> concatenate3/128
